simulink model "GFo_29bus"  (R2017b)
settings: Solver=ode1  StartTime=0.0  StopTime=4.5  FixedStep=Time_Step  RelTol=1e-3  EnableMultiTasking=on
PreLoadFcn:
  | Init_29bus;
InitFcn:
  | Init_29bus;
undefined symbols (not defined in the file): D1, D11, Delta, Time_Step, VSC01_Delta_P_Time_Step, VSC01_Delta_P_Value
libraries: powerlib x168, sps_avr x6, GFo_Lib x1
(part 2 of 5)

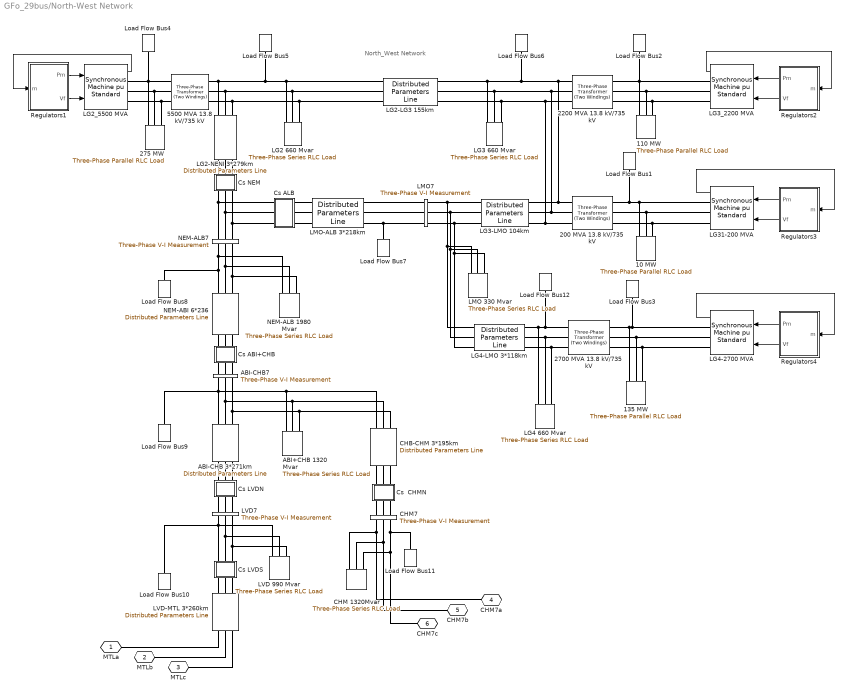
== system GFo_29bus/North-West Network ==
  note: North_West Network
  10 MW : powerlib/Elements/Three-Phase Parallel RLC Load  LConnTagsString=A|B|C  Configuration=Y (grounded)  NominalVoltage=(13800)*1  Vabc=[1e3 1e3 1e3]  Vabcp=[1e3 1e3 1e3]  NominalFrequency=60  UnbalancedPower=off  ActivePower=10000000  InductivePower=0  CapacitivePower=0  Pabc=[10e3 9e3 11e3]  QLabc=[100 90 110]  QCabc=[100 90 110]  Pabcp=[10e3 9e3 11e3]  QLabcp=[100 90 110]  QCabcp=[100 90 110]  Measurements=None  LoadType=constant PQ
  110 MW : powerlib/Elements/Three-Phase Parallel RLC Load  LConnTagsString=A|B|C  Configuration=Y (grounded)  NominalVoltage=(13800)*1  Vabc=[1e3 1e3 1e3]  Vabcp=[1e3 1e3 1e3]  NominalFrequency=60  UnbalancedPower=off  ActivePower=110000000  InductivePower=0  CapacitivePower=0  Pabc=[10e3 9e3 11e3]  QLabc=[100 90 110]  QCabc=[100 90 110]  Pabcp=[10e3 9e3 11e3]  QLabcp=[100 90 110]  QCabcp=[100 90 110]  Measurements=None  LoadType=constant PQ
  135 MW : powerlib/Elements/Three-Phase Parallel RLC Load  LConnTagsString=A|B|C  Configuration=Y (grounded)  NominalVoltage=(13800)*1  Vabc=[1e3 1e3 1e3]  Vabcp=[1e3 1e3 1e3]  NominalFrequency=60  UnbalancedPower=off  ActivePower=135000000  InductivePower=0  CapacitivePower=0  Pabc=[10e3 9e3 11e3]  QLabc=[100 90 110]  QCabc=[100 90 110]  Pabcp=[10e3 9e3 11e3]  QLabcp=[100 90 110]  QCabcp=[100 90 110]  Measurements=None  LoadType=constant PQ
  200 MVA 13.8 kV/735 kV : powerlib/Elements/Three-Phase Transformer (Two Windings)  Winding1Connection=Delta (D1)  Winding2Connection=Yg  CoreType=Three single-phase transformers  SetSaturation=off  Hysteresis=off  DataFile='basic_model'  SetInitialFlux=off  Measurements=None  UNITS=pu  NominalPower=[ 200e6 60 ]  Winding1="[ 13.8e3 0.002  0.0]"  Winding2=[ 735e3 0.002 0.12]  Rm=500  Lm=500  L0=0.5  Saturation="[ 0,0  ;  0.005,1.2  ;  1.0,1.4 ]"  InitialFluxes=[ 0.8 , -0.8 , 0.7 ]  MoreParameters=off  BreakLoop=off  DataType=off  TransfoNumber=0
  2200 MVA 13.8 kV/735 kV : powerlib/Elements/Three-Phase Transformer (Two Windings)  Winding1Connection=Delta (D1)  Winding2Connection=Yg  CoreType=Three single-phase transformers  SetSaturation=off  Hysteresis=off  DataFile='basic_model'  SetInitialFlux=off  Measurements=None  UNITS=pu  NominalPower=[ 2200e6 60 ]  Winding1="[ 13.8e3 0.002  0.0]"  Winding2=[ 735e3 0.002 0.12]  Rm=500  Lm=500  L0=0.5  Saturation="[ 0,0  ;  0.005,1.2  ;  1.0,1.4 ]"  InitialFluxes=[ 0.8 , -0.8 , 0.7 ]  MoreParameters=off  BreakLoop=off  DataType=off  TransfoNumber=0
  2700 MVA 13.8 kV/735 kV : powerlib/Elements/Three-Phase Transformer (Two Windings)  Winding1Connection=Delta (D1)  Winding2Connection=Yg  CoreType=Three single-phase transformers  SetSaturation=off  Hysteresis=off  DataFile='basic_model'  SetInitialFlux=off  Measurements=None  UNITS=pu  NominalPower=[ 2700e6 60 ]  Winding1="[ 13.8e3 0.002  0.0]"  Winding2=[ 735e3 0.002 0.12]  Rm=500  Lm=500  L0=0.5  Saturation="[ 0,0  ;  0.005,1.2  ;  1.0,1.4 ]"  InitialFluxes=[ 0.8 , -0.8 , 0.7 ]  MoreParameters=off  BreakLoop=off  DataType=off  TransfoNumber=0
  275 MW : powerlib/Elements/Three-Phase Parallel RLC Load  LConnTagsString=A|B|C  Configuration=Y (grounded)  NominalVoltage=(13800)*1  Vabc=[1e3 1e3 1e3]  Vabcp=[1e3 1e3 1e3]  NominalFrequency=60  UnbalancedPower=off  ActivePower=275000000  InductivePower=0  CapacitivePower=0  Pabc=[10e3 9e3 11e3]  QLabc=[100 90 110]  QCabc=[100 90 110]  Pabcp=[10e3 9e3 11e3]  QLabcp=[100 90 110]  QCabcp=[100 90 110]  Measurements=None  LoadType=constant PQ
  5500 MVA 13.8 kV/735 kV : powerlib/Elements/Three-Phase Transformer (Two Windings)  Winding1Connection=Delta (D1)  Winding2Connection=Yg  CoreType=Three single-phase transformers  SetSaturation=off  Hysteresis=off  DataFile='basic_model'  SetInitialFlux=off  Measurements=None  UNITS=pu  NominalPower=[ 5500e6 60 ]  Winding1="[ 13.8e3 0.002  0.0]"  Winding2=[ 735e3 0.002 0.12]  Rm=500  Lm=500  L0=0.5  Saturation="[ 0,0  ;  0.005,1.2  ;  1.0,1.4 ]"  InitialFluxes=[ 0.8 , -0.8 , 0.7 ]  MoreParameters=off  BreakLoop=off  DataType=off  TransfoNumber=0
  ABI+CHB 1320 Mvar : powerlib/Elements/Three-Phase Series RLC Load  LConnTagsString=A|B|C  Configuration=Y (grounded)  NominalVoltage=735e3  Vabc=[1e3 1e3 1e3]  Vabcp=[1e3 1e3 1e3]  NominalFrequency=60  UnbalancedPower=off  ActivePower=4400000  InductivePower=1320e6  CapacitivePower=0  Pabc=[10e3 9e3 11e3]  QLabc=[100 90 110]  QCabc=[100 90 110]  Pabcp=[10e3 9e3 11e3]  QLabcp=[100 90 110]  QCabcp=[100 90 110]  Measurements=None  LoadType=constant Z
  ABI-CHB 3*271km : powerlib/Elements/Distributed Parameters Line  Phases=3  Frequency=60  Resistance="[0.01273  0.3864]/3"  Inductance="[0.9337e-3  4.1264e-3]/3"  Capacitance=[12.74e-9 7.751e-9]*3  Length=271  x1=[-0.00156 -3.8452560916682e-08 0 0;-0.00152 -3.64189744128759e-08 0 0;-0.00148 -3.43771065483522e-08 0 0;-0.00144 -3.2327421626255e-08 0 0;-0.0014 -3.02703857272598e-08 0 0;-0.00136 -2.82064666035909e-08 0 0;-0.00132 -2.61361335726585e-08 0 0;-0.00128 -2.40598574103402e-08 0 0;-0.00124 -2.19781102439301e-08 0 0;-0.0012 -1.98913654447816e-08 0 0;-0.00116 -1.78000975206669e-08 0 0;-0.00112 -1.57047820078775e-08 0 0;-0.00108 -1.36058953630917e-08 0 0;-0.00104 -1.15039148550326e-08 0 0;-0.001 -9.39931845594105e-09 0 0;-0.00096 -7.29258473288888e-09 123121.325667195 -796454.043668796;-0.00092 -5.18419273895701e-09 135117.082377557 -794506.987955466;-0.00088 -3.07462190430287e-09 147082.114628586 -792379.268204613;-0.00084 -9.6435192714211e-10 159013.701675131 -790071.368241357;-0.0008 1.14613733533067e-09 170909.130377191 -787583.812862248;-0.00076 3.25636597605726e-09 182765.69581686 -784917.167715928;-0.00072 5.3658541472426e-09 194580.701913405 -782072.039174507;-0.00068 7.47412216946802e-09 206351.462036328 -779049.07419568;-0.00064 9.58069064076618e-09 218075.299616282 -775848.960175613;-0.0006 1.1685080545633e-08 229749.548753705 -772472.424792639;-0.00056 1.37868133639516e-08 241371.554825018 -768920.235841786;-0.00052 1.58854111798036e-08 252938.675086262 -765193.201060188;-0.00048 1.79803967901433e-08 264448.279274042 -761292.167943414;-0.00044 2.00712938133092e-08 275897.750203621 -757218.023552754;-0.0004 2.21576267973495e-08 287284.484364043 -752971.694313508;-0.00036 2.42389213281353e-08 298605.892510158 -748554.145804326;-0.00032 2.63147041372386e-08 309859.400251383 -743966.382537645;-0.00028 2.83845032095495e-08 321042.448637104 -739209.447731267;-0.00024 3.0447847890608e-08 332152.494738558 -734284.423071146;-0.0002 3.25042689936273e-08 343187.012227069 -729192.428465418;-0.00016 3.45532989061823e-08 354143.491948518 -723934.621789744;-0.00012 3.6594471696541e-08 365019.442493902 -718512.198624022;-8e-05 3.86273232196132e-08 375812.390765856 -712926.391980518;-4e-05 4.0651391222493e-08 386519.882541018 -707178.472023493]  x2=[-0.00156 -7.69394572937684e-08 0 0;-0.00152 -7.25740724890193e-08 0 0;-0.00148 -6.81921849660384e-08 0 0;-0.00144 -6.37947911282605e-08 0 0;-0.0014 -5.93828909051229e-08 0 0;-0.00136 -5.49574875246898e-08 0 0;-0.00132 -5.05195872855267e-08 0 0;-0.00128 -4.60701993278772e-08 0 0;-0.00124 -4.16103354041931e-08 0 0;-0.0012 -3.71410096490703e-08 0 0;-0.00116 -3.26632383486437e-08 0 0;-0.00112 -2.81780397094924e-08 0 0;-0.00108 -2.36864336271083e-08 0 0;-0.00104 -1.91894414539804e-08 0 0;-0.001 -1.46880857673486e-08 0 0;-0.00096 -1.0183390136678e-08 -123389.155033361 -813372.162639077;-0.00092 -5.67637889090808e-09 -111110.252745338 -815140.324111655;-0.00088 -1.16807688552937e-09 -98806.084944014 -816723.129704001;-0.00084 3.34049073046001e-09 -86479.4494910415 -818120.219499772;-0.0008 7.84829874766446e-09 -74133.1493570218 -819331.275812798;-0.00076 1.23543221294145e-08 -61769.9919841353 -820356.023259316;-0.00072 1.68575362448515e-08 -49392.7886477534 -821194.228820593;-0.00068 2.13569171019196e-08 -37004.3538171782 -821845.701895914;-0.00064 2.5851441580213e-08 -24607.504515657 -822310.29434592;-0.0006 3.03400876636243e-08 -12205.059679815 -822587.900526293;-0.00056 3.48218346727427e-08 200.160481346233 -822678.457311783;-0.00052 3.92956634969472e-08 12605.3351277401 -822581.944110556;-0.00048 4.37605568261439e-08 25007.6434296298 -822298.382868884;-0.00044 4.82154993820933e-08 37404.2652090602 -821827.838066146;-0.0004 5.2659478149276e-08 49792.3815811428 -821170.416700174;-0.00036 5.70914826052435e-08 62169.175595045 -820326.268262915;-0.00032 6.15105049504026e-08 74531.8328745411 -819295.584706447;-0.00028 6.59155403371799e-08 86877.5422579766 -818078.60039932;-0.00024 7.0305587098516e-08 99203.4964375027 -816675.592073272;-0.0002 7.46796469756355e-08 111506.892597433 -815086.878760297;-0.00016 7.90367253450425e-08 123784.933051582 -813312.821720102;-0.00012 8.33758314446898e-08 136034.82587943 -811353.824357958;-8e-05 8.7695978599269e-08 148253.785560988 -809210.332132973;-4e-05 9.19961844445728e-08 160439.033610196 -806882.832456794]  x3=[-0.00156 -1.37891885995195e-09 0 0;-0.00152 -1.3722422723815e-09 0 0;-0.00148 -1.36525364875204e-09 0 0;-0.00144 -1.35795457821629e-09 0 0;-0.0014 -1.35034672051995e-09 0 0;-0.00136 -1.34243180562426e-09 0 0;-0.00132 -1.33421163331262e-09 0 0;-0.00128 -1.32568807278131e-09 0 0;-0.00124 -1.31686306221449e-09 0 0;-0.0012 -1.30773860834347e-09 0 0;-0.00116 -1.29831678599038e-09 0 0;-0.00112 -1.28859973759635e-09 0 0;-0.00108 -1.27858967273441e-09 0 0;-0.00104 -1.26828886760697e-09 0 0;-0.001 -1.2576996645283e-09 0 0;-0.00096 -1.24682447139185e-09 -1025.79722603647 -1146.3924319426;-0.00092 -1.23566576112277e-09 -1008.39460171361 -1161.73052146923;-0.00088 -1.22422607111553e-09 -990.762677154345 -1176.80444349362;-0.00084 -1.212508002657e-09 -972.90546170627 -1191.61077033589;-0.0008 -1.20051422033489e-09 -954.827015946182 -1206.146135165;-0.00076 -1.18824745143186e-09 -936.531450756745 -1220.40723276433;-0.00072 -1.17571048530539e-09 -918.02292639171 -1234.39082028327;-0.00068 -1.16290617275346e-09 -899.305651529905 -1248.09371797462;-0.00064 -1.14983742536632e-09 -880.383882318225 -1261.5128099176;-0.0006 -1.13650721486443e-09 -861.261921403812 -1274.64504472642;-0.00056 -1.1229185724227e-09 -841.944116955679 -1287.48743624415;-0.00052 -1.10907458798123e-09 -822.434861675967 -1300.03706422169;-0.00048 -1.09497840954271e-09 -802.738591801085 -1312.29107498188;-0.00044 -1.08063324245656e-09 -782.859786092952 -1324.24668206832;-0.0004 -1.06604234869005e-09 -762.802964820555 -1335.90116687908;-0.00036 -1.05120904608661e-09 -742.572688732092 -1347.25187928482;-0.00032 -1.03613670761132e-09 -722.173558017884 -1358.29623823141;-0.00028 -1.02082876058399e-09 -701.610211264343 -1369.03173232688;-0.00024 -1.00528868589976e-09 -680.88732439919 -1379.45592041244;-0.0002 -9.89520017237592e-10 -660.00960962819 -1389.56643211762;-0.00016 -9.73526340256762e-10 -638.981814363641 -1399.36096839924;-0.00012 -9.57311291781491e-10 -617.80872014485 -1408.83730206423;-8e-05 -9.40878558973969e-10 -596.495141550854 -1417.99327827602;-4e-05 -9.24231878495929e-10 -575.045925105624 -1426.82681504459]  x4=[-0.00156 4.69352936032902e-10 0 0;-0.00152 4.84294936998338e-10 0 0;-0.00148 4.99126813471482e-10 0 0;-0.00144 5.13845192811529e-10 0 0;-0.0014 5.28446728185943e-10 0 0;-0.00136 5.42928099331498e-10 0 0;-0.00132 5.57286013309277e-10 0 0;-0.00128 5.7151720525346e-10 0 0;-0.00124 5.85618439113723e-10 0 0;-0.0012 5.99586508391089e-10 0 0;-0.00116 6.13418236867062e-10 0 0;-0.00112 6.27110479325864e-10 0 0;-0.00108 6.40660122269638e-10 0 0;-0.00104 6.54064084626425e-10 0 0;-0.001 6.67319318450777e-10 0 0;-0.00096 6.8042280961683e-10 -2132.85907292929 -16521.1252471031;-0.00092 6.93371578503692e-10 -1883.49323206401 -16551.4092311591;-0.00088 7.06162680672985e-10 -1633.69910108033 -16577.9295674892;-0.00084 7.1879320753838e-10 -1383.53348100947 -16600.6802255976;-0.0008 7.31260287026989e-10 -1133.05325735612 -16619.6560321809;-0.00076 7.43561084232449e-10 -882.315387163084 -16634.8526723043;-0.00072 7.55692802059552e-10 -631.376886059769 -16646.2666903828;-0.00068 7.67652681860283e-10 -380.294815297326 -16653.8954909673;-0.00064 7.79438004061115e-10 -129.126268773408 -16657.7373393341;-0.0006 7.9104608878141e-10 122.071639950492 -16657.7913618803;-0.00056 8.02474296442807e-10 373.241790636168 -16654.0575463214;-0.00052 8.13720028369436e-10 624.327069357354 -16646.5367416949;-0.00048 8.24780727378837e-10 875.270381486935 -16635.230658167;-0.00044 8.35653878363439e-10 1126.01466467978 -16620.1418666436;-0.0004 8.46337008862472e-10 1376.50290184821 -16601.2737981857;-0.00036 8.5682768962419e-10 1626.67813412721 -16578.6307432293;-0.00032 8.67123535158254e-10 1876.48347382639 -16552.21785061;-0.00028 8.77222204278178e-10 2125.86211736573 -16522.0411263917;-0.00024 8.87121400633692e-10 2374.75735819223 -16488.1074325012;-0.0002 8.9681887323291e-10 2623.11259967451 -16450.424485168;-0.00016 9.06312416954192e-10 2870.87136797239 -16409.0008531693;-0.00012 9.15599873047564e-10 3117.97732487853 -16363.8459558818;-8e-05 9.24679129625602e-10 3364.37428062928 -16314.9700611397;-4e-05 9.33548122143656e-10 3610.00620668175 -16262.3842829]  x5=0.00153261764655846  V1=ones(3,3)  V2=ones(3,3)  I1=ones(3,3)  I2=ones(3,3)  nHarmo=1  Measurements=None
      settings: AttributesFormatString=\n  SourceProductName=Simscape Power Systems
  ABI-CHB7 : powerlib/Measurements/Three-Phase V-I Measurement  VoltageMeasurement=no  SetLabelV=on  LabelV=Vabc_ABI7  Vpu=on  VpuLL=off  CurrentMeasurement=no  SetLabelI=off  LabelI=A1  Ipu=off  Pbase=100e6  Vbase=500e3  OutputType=Magnitude  PhasorSimulation=off  PSBequivalent=0
  CHB-CHM 3*195km : powerlib/Elements/Distributed Parameters Line  Phases=3  Frequency=60  Resistance="[0.01273  0.3864]/3"  Inductance="[0.9337e-3  4.1264e-3]/3"  Capacitance=[12.74e-9 7.751e-9]*3  Length=195  x1=[-0.00112 -1.57340244697438e-08 0 0;-0.00108 -1.36362948191761e-08 0 0;-0.00104 -1.15354643927609e-08 0 0;-0.001 -9.43201090122036e-09 0 0;-0.00096 -7.32641265173913e-09 0 0;-0.00092 -5.21914843920118e-09 0 0;-0.00088 -3.11069743731617e-09 0 0;-0.00084 -1.00153908965942e-09 0 0;-0.0008 1.1078469993494e-09 0 0;-0.00076 3.21698117350424e-09 0 0;-0.00072 5.32538383388229e-09 0 0;-0.00068 7.43257554790067e-09 206351.462036328 -779049.07419568;-0.00064 9.53807715833526e-09 218075.299616282 -775848.960175613;-0.0006 1.16414098922769e-08 229749.548753705 -772472.424792639;-0.00056 1.37420954700003e-08 241371.554825018 -768920.235841786;-0.00052 1.58396562137206e-08 252938.675086262 -765193.201060188;-0.00048 1.79336151562133e-08 264448.279274042 -761292.167943414;-0.00044 2.00234961492724e-08 275897.750203621 -757218.023552754;-0.0004 2.21088239719824e-08 287284.484364043 -752971.694313508;-0.00036 2.41891244387795e-08 298605.892510158 -748554.145804326;-0.00032 2.62639245072774e-08 309859.400251383 -743966.382537645;-0.00028 2.83327523858328e-08 321042.448637104 -739209.447731267;-0.00024 3.03951376408269e-08 332152.494738558 -734284.423071146;-0.0002 3.24506113036379e-08 343187.012227069 -729192.428465418;-0.00016 3.44987059772807e-08 354143.491948518 -723934.621789744;-0.00012 3.65389559426884e-08 365019.442493902 -718512.198624022;-8e-05 3.85708972646133e-08 375812.390765856 -712926.391980518;-4e-05 4.05940678971215e-08 386519.882541018 -707178.472023493]  x2=[-0.00112 -6.77914093750269e-09 0 0;-0.00108 -5.32034013604767e-09 0 0;-0.00104 -3.86032953512641e-09 0 0;-0.001 -2.3994411285589e-09 0 0;-0.00096 -9.38007109770666e-10 0 0;-0.00092 5.23640203745304e-10 0 0;-0.00088 1.98516844599463e-09 0 0;-0.00084 3.4462452780587e-09 0 0;-0.0008 4.90653846366568e-09 0 0;-0.00076 6.36571594473822e-09 0 0;-0.00072 7.82344591690052e-09 0 0;-0.00068 9.27939690492784e-09 118695.788002337 -793597.57910968;-0.00064 1.07332378381211e-08 130648.969041902 -791717.567766348;-0.0006 1.21846381255895e-08 142572.441632576 -789657.526675586;-0.00056 1.36332677314239e-08 154463.494479515 -787417.924272976;-0.00052 1.50787972497445e-08 166319.423659846 -784999.269824789;-0.00048 1.65208979796045e-08 178137.533237514 -782402.113312189;-0.00044 1.79592419997342e-08 189915.135876316 -779627.04530617;-0.0004 1.9393502243107e-08 201649.553450979 -776674.696833266;-0.00036 2.08233525713121e-08 213338.117656138 -773545.739232059;-0.00032 2.22484678487155e-08 224978.170613092 -770240.884000526;-0.00028 2.36685240163927e-08 236567.065474178 -766760.882634245;-0.00024 2.50831981658172e-08 248102.167024643 -763106.526455517;-0.0002 2.64921686122871e-08 259580.852281868 -759278.646433424;-0.00016 2.78951149680733e-08 271000.511091814 -755278.112994872;-0.00012 2.9291718215273e-08 282358.546722546 -751105.835826666;-8e-05 3.06816607783516e-08 293652.376454711 -746762.763668654;-4e-05 3.20646265963565e-08 304879.432168819 -742249.884097991]  x3=[-0.00112 2.33399313420562e-10 0 0;-0.00108 2.41014554085093e-10 0 0;-0.00104 2.48574990118446e-10 0 0;-0.001 2.56078902342666e-10 0 0;-0.00096 2.63524584432823e-10 0 0;-0.00092 2.7091034330502e-10 0 0;-0.00088 2.7823449950138e-10 0 0;-0.00084 2.85495387571946e-10 0 0;-0.0008 2.92691356453385e-10 0 0;-0.00076 2.9982076984443e-10 0 0;-0.00072 3.06882006577956e-10 0 0;-0.00068 3.13873460989624e-10 399.328451062111 -5036.75917956306;-0.00064 3.20793543282992e-10 475.231927360191 -5030.16562723451;-0.0006 3.27640679891024e-10 551.027340016215 -5022.42825862063;-0.00056 3.34413313833901e-10 626.697453806977 -5013.54883313232;-0.00052 3.4110990507307e-10 702.225062001152 -5003.52936987436;-0.00048 3.47728930861432e-10 777.592990271958 -4992.37214718629;-0.00044 3.54268886089603e-10 852.784100602454 -4980.07970212433;-0.0004 3.60728283628161e-10 927.781295182568 -4966.65482988449;-0.00036 3.67105654665811e-10 1002.567520297 -4952.10058316694;-0.00032 3.73399549043374e-10 1077.1257702031 -4936.42027148187;-0.00028 3.79608535583546e-10 1151.43909099779 -4919.61746039695;-0.00024 3.8573120241633e-10 1225.49058447277 -4901.6959707265;-0.0002 3.91766157300088e-10 1299.26341195702 -4882.65987766274;-0.00016 3.97712027938125e-10 1372.74079814577 -4862.51350984906;-0.00012 4.0356746229073e-10 1445.90603491502 -4841.26144839577;-8e-05 4.09331128882629e-10 1518.74248512091 -4818.90852583838;-4e-05 4.1500171710574e-10 1591.23358638275 -4795.45982503871]  x4=[-0.00112 -5.12172901448853e-10 0 0;-0.00108 -5.06547662638855e-10 0 0;-0.00104 -5.00807239258654e-10 0 0;-0.001 -4.94952936631024e-10 0 0;-0.00096 -4.88986085973895e-10 0 0;-0.00092 -4.82908044097653e-10 0 0;-0.00088 -4.76720193096604e-10 0 0;-0.00084 -4.70423940034705e-10 0 0;-0.0008 -4.64020716625606e-10 0 0;-0.00076 -4.57511978907089e-10 0 0;-0.00072 -4.50899206909985e-10 0 0;-0.00068 -4.44183904321619e-10 966.84418643773 -12727.6275437189;-0.00064 -4.37367598143889e-10 1158.65512674327 -12711.6018358708;-0.0006 -4.30451838346038e-10 1350.2025988648 -12692.6856193854;-0.00056 -4.23438197512206e-10 1541.443046559 -12670.8831956472;-0.00052 -4.16328270483835e-10 1732.33298339725 -12646.1995223393;-0.00048 -4.09123673997018e-10 1922.82900265409 -12618.6402123163;-0.00044 -4.01826046314867e-10 2112.88778717749 -12588.2115323274;-0.0004 -3.94437046854984e-10 2302.46611923885 -12554.9204015923;-0.00036 -3.86958355812126e-10 2491.52089036032 -12518.7743902268;-0.00032 -3.79391673776144e-10 2680.00911111728 -12479.7817175223;-0.00028 -3.71738721345279e-10 2867.88792091379 -12437.9512500763;-0.00024 -3.64001238734918e-10 3055.1145977287 -12393.2924997764;-0.0002 -3.56180985381882e-10 3241.64656783027 -12345.8156216372;-0.00016 -3.48279739544345e-10 3427.44141545708 -12295.5314114914;-0.00012 -3.40299297897471e-10 3612.45689246302 -12242.4513035349;-8e-05 -3.32241475124872e-10 3796.65092792411 -12186.5873677262;-4e-05 -3.24108103505957e-10 3979.98163770511 -12127.9523070429]  x5=0.0011028060556417  V1=ones(3,3)  V2=ones(3,3)  I1=ones(3,3)  I2=ones(3,3)  nHarmo=1  Measurements=None
      settings: AttributesFormatString=\n  SourceProductName=Simscape Power Systems
  CHM 1320Mvar : powerlib/Elements/Three-Phase Series RLC Load  LConnTagsString=A|B|C  Configuration=Y (grounded)  NominalVoltage=735e3  Vabc=[1e3 1e3 1e3]  Vabcp=[1e3 1e3 1e3]  NominalFrequency=60  UnbalancedPower=off  ActivePower=4400000  InductivePower=1320e6  CapacitivePower=0  Pabc=[10e3 9e3 11e3]  QLabc=[100 90 110]  QCabc=[100 90 110]  Pabcp=[10e3 9e3 11e3]  QLabcp=[100 90 110]  QCabcp=[100 90 110]  Measurements=None  LoadType=constant Z
  CHM7 : powerlib/Measurements/Three-Phase V-I Measurement  VoltageMeasurement=no  SetLabelV=on  LabelV=Vabc_CHM7  Vpu=on  VpuLL=off  CurrentMeasurement=no  SetLabelI=off  LabelI=A1  Ipu=off  Pbase=100e6  Vbase=735e3  OutputType=Magnitude  PhasorSimulation=off  PSBequivalent=0
  "Cs  CHMN " : Subsystem  mask{Xc=25/3}
      mask prompts: Xc "Condensator Reactance at  60Hz  (ohm):"
      mask help: Series Compensation
      mask init:
      | Cs=1/Xc/(2*pi*60);
      mask Display: disp('Cs')
  "Cs ABI+CHB " : Subsystem  mask{Xc=25/6}
      mask prompts: Xc "Condensator Reactance at  60Hz  (ohm):"
      mask help: Series Compensation
      mask init:
      | Cs=1/Xc/(2*pi*60);
      mask Display: disp('Cs')
  Cs ALB : Subsystem  mask{Xc=16/3}
      mask prompts: Xc "Reactance @ 60Hz du condensateur (ohm):"
      mask init:
      | Cs=1/Xc/(2*pi*60);
      mask Display: disp('Cs')
  "Cs LVDN " : Subsystem  mask{Xc=34/3}
      mask prompts: Xc "Condensator Reactance at  60Hz  (ohm):"
      mask help: Series Compensation
      mask init:
      | Cs=1/Xc/(2*pi*60);
      mask Display: disp('Cs')
  "Cs LVDS " : Subsystem  mask{Xc=34/3}
      mask prompts: Xc "Condensator Reactance at  60Hz  (ohm):"
      mask help: Series Compensation
      mask init:
      | Cs=1/Xc/(2*pi*60);
      mask Display: disp('Cs')
  "Cs NEM " : Subsystem  mask{Xc=16/3}
      mask prompts: Xc "Condensator Reactance at  60Hz  (ohm):"
      mask help: Series Compensation
      mask init:
      | Cs=1/Xc/(2*pi*60);
      mask Display: disp('Cs')
  LG2 660 Mvar : powerlib/Elements/Three-Phase Series RLC Load  LConnTagsString=A|B|C  Configuration=Y (grounded)  NominalVoltage=735e3  Vabc=[1e3 1e3 1e3]  Vabcp=[1e3 1e3 1e3]  NominalFrequency=60  UnbalancedPower=off  ActivePower=2200000  InductivePower=660e6  CapacitivePower=0  Pabc=[10e3 9e3 11e3]  QLabc=[100 90 110]  QCabc=[100 90 110]  Pabcp=[10e3 9e3 11e3]  QLabcp=[100 90 110]  QCabcp=[100 90 110]  Measurements=None  LoadType=constant Z
  LG2-LG3 155km : powerlib/Elements/Distributed Parameters Line  Phases=3  Frequency=60  Resistance="[0.01273  0.3864]"  Inductance="[0.9337e-3  4.1264e-3]"  Capacitance=[12.74e-9 7.751e-9]  Length=155  x1=[-0.00088 -1.9399100123935e-09 415587.672863184 -614459.217668148;-0.00084 -1.83186752142981e-09 424805.862965605 -608122.737717224;-0.0008 -1.72340847958909e-09 433927.455878156 -601647.975899972;-0.00076 -1.61455754952216e-09 442950.377429272 -595036.40452139;-0.00072 -1.50533948299182e-09 451872.575884402 -588289.526995796;-0.00068 -1.39577911524454e-09 460692.022412559 -581408.877504956;-0.00064 -1.28590135936314e-09 469406.711547658 -574396.020649228;-0.0006 -1.17573120060176e-09 478014.661644543 -567252.551091784;-0.00056 -1.06529369070444e-09 486513.915329592 -559980.093196;-0.00052 -9.54613942208553e-10 494902.539945812 -552580.300656086;-0.00048 -8.43717122734449e-10 503178.627992307 -545054.856121052;-0.00044 -7.32628449262542e-10 511340.297558024 -537405.470812089;-0.0004 -6.21373182399191e-10 519385.692749687 -529633.884133451;-0.00036 -5.09976620632657e-10 527312.98411381 -521741.863276929;-0.00032 -3.98464094580442e-10 535120.369052699 -513731.202820008;-0.00028 -2.86860961229327e-10 542806.072234347 -505603.724317795;-0.00024 -1.75192598169412e-10 550368.34599613 -497361.275888813;-0.0002 -6.34843978234705e-11 557805.470742207 -489005.731794755;-0.00016 4.82382383270702e-11 565115.755334547 -480538.992014292;-0.00012 1.59949905518204e-10 572297.537477475 -471962.981811038;-8e-05 2.71625201480173e-10 579349.184095664 -463279.651295754;-4e-05 3.8323873221372e-10 586269.091705484 -454490.97498292]  x2=[-0.00088 -2.93952786722991e-09 413310.722035332 -609787.007539505;-0.00084 -2.90618950351965e-09 422458.718213806 -603485.390922945;-0.0008 -2.87219029737821e-09 431510.650922886 -597046.546932726;-0.00076 -2.83753797993185e-09 440464.461831136 -590471.939706444;-0.00072 -2.80224043081874e-09 449318.114919169 -583763.064253086;-0.00068 -2.76630567639716e-09 458069.596942624 -576921.446113075;-0.00064 -2.72974188792036e-09 466716.917889958 -569948.641011377;-0.0006 -2.69255737967855e-09 475258.111434959 -562846.234503741;-0.00056 -2.65476060710822e-09 483691.235383871 -555615.841616157;-0.00052 -2.61636016486952e-09 492014.372117033 -548259.106477617;-0.00048 -2.57736478489185e-09 500225.629024926 -540777.701946249;-0.00044 -2.53778333438835e-09 508323.138938541 -533173.329228927;-0.0004 -2.49762481383952e-09 516305.060553954 -525447.717494429;-0.00036 -2.45689835494662e-09 524169.578851022 -517602.623480241;-0.00032 -2.4156132185552e-09 531914.905506105 -509639.831093089;-0.00028 -2.37377879254923e-09 539539.279298715 -501561.151003293;-0.00024 -2.33140458971644e-09 547040.966512001 -493368.420233037;-0.0002 -2.28850024558512e-09 554418.261326982 -485063.501738649;-0.00016 -2.24507551623315e-09 561669.486210437 -476648.283986975;-0.00012 -2.20114027606948e-09 568792.992296359 -468124.680525962;-8e-05 -2.15670451558887e-09 575787.159760895 -459494.629549533;-4e-05 -2.11177833910004e-09 582650.398190678 -450760.093456857]  x3=[-0.00088 1.40286124984699e-11 1382.36701026453 -2367.08434783059;-0.00084 1.40500137891377e-11 1417.90313254797 -2345.97063689771;-0.0008 1.4068220227832e-11 1453.11683588655 -2324.32347247279;-0.00076 1.40832276745657e-11 1488.00011298779 -2302.14777693433;-0.00072 1.40950327167747e-11 1522.54503169531 -2279.44859284429;-0.00068 1.41036326700944e-11 1556.74373679248 -2256.23108180135;-0.00064 1.41090255789694e-11 1590.5884517887 -2232.50052326732;-0.0006 1.41112102170988e-11 1624.07148068763 -2208.26231336657;-0.00056 1.41101860877147e-11 1657.18520973725 -2183.521963659;-0.00052 1.41059534236954e-11 1689.92210916113 -2158.28509988678;-0.00048 1.4098513187512e-11 1722.27473487065 -2132.55746069511;-0.00044 1.40878670710103e-11 1754.23573015773 -2106.34489632727;-0.0004 1.40740174950251e-11 1785.79782736766 -2079.65336729434;-0.00036 1.40569676088308e-11 1816.95384955171 -2052.48894301987;-0.00032 1.40367212894243e-11 1847.69671209911 -2024.85780045966;-0.00028 1.40132831406442e-11 1878.01942434804 -1996.76622269725;-0.00024 1.39866584921233e-11 1907.91509117522 -1968.22059751518;-0.0002 1.3956853398077e-11 1937.37691456383 -1939.22741594245;-0.00016 1.39238746359268e-11 1966.39819514929 -1909.79327077852;-0.00012 1.38877297047588e-11 1994.97233374267 -1879.92485509417;-8e-05 1.38484268236187e-11 2023.09283283127 -1849.62896070956;-4e-05 1.38059749296425e-11 2050.75329805609 -1818.91247664979]  x4=[-0.00088 -2.31758602658944e-11 1207.15321374292 -2438.84076514513;-0.00084 -2.30254032880232e-11 1243.79135626553 -2420.36094489669;-0.0008 -2.28697105320071e-11 1280.14667135972 -2401.33075544169;-0.00076 -2.27088174010359e-11 1316.21089214036 -2381.75452408109;-0.00072 -2.25427604808202e-11 1351.97581791464 -2361.63670228109;-0.00068 -2.23715775312717e-11 1387.43331604688 -2340.98186466088;-0.00064 -2.21953074779168e-11 1422.57532380776 -2319.79470795242;-0.0006 -2.20139904030456e-11 1457.39385020777 -2298.08004993242;-0.00056 -2.18276675365974e-11 1491.88097781428 -2275.84282832687;-0.00052 -2.16363812467851e-11 1526.02886455186 -2253.08809968819;-0.00048 -2.14401750304615e-11 1559.82974548556 -2229.82103824544;-0.00044 -2.12390935032282e-11 1593.27593458653 -2206.04693472775;-0.0004 -2.10331823892903e-11 1626.35982647981 -2181.77119516125;-0.00036 -2.08224885110596e-11 1659.07389817367 -2156.99933963976;-0.00032 -2.0607059778507e-11 1691.41071077033 -2131.7370010696;-0.00028 -2.03869451782684e-11 1723.36291115747 -2105.98992388872;-0.00024 -2.01621947625059e-11 1754.92323368026 -2079.76396276043;-0.0002 -1.99328596375257e-11 1786.08450179352 -2053.06508124213;-0.00016 -1.96989919521576e-11 1816.83962969362 -2025.89935042924;-0.00012 -1.94606448858964e-11 1847.18162392967 -1998.27294757467;-8e-05 -1.92178726368097e-11 1877.10358499387 -1970.19215468419;-4e-05 -1.89707304092132e-11 1906.59870889028 -1941.66335708795]  x5=0.000876589428843401  V1=ones(3,3)  V2=ones(3,3)  I1=ones(3,3)  I2=ones(3,3)  nHarmo=1  Measurements=None
      settings: AttributesFormatString=\n  SourceProductName=Simscape Power Systems
  LG2-NENI 3*279km : powerlib/Elements/Distributed Parameters Line  Phases=3  Frequency=60  Resistance="[0.01273  0.3864]/3"  Inductance="[0.9337e-3  4.1264e-3]/3"  Capacitance=[12.74e-9 7.751e-9]*3  Length=279  x1=[-0.0016 -3.78600842431516e-09 0 0;-0.00156 -3.68954651697759e-09 0 0;-0.00152 -3.59224563857934e-09 0 0;-0.00148 -3.4941279145011e-09 0 0;-0.00144 -3.39521565586717e-09 0 0;-0.0014 -3.29553135447219e-09 0 0;-0.00136 -3.19509767766665e-09 0 0;-0.00132 -3.09393746320256e-09 0 0;-0.00128 -2.99207371404032e-09 0 0;-0.00124 -2.88952959311806e-09 0 0;-0.0012 -2.78632841808456e-09 0 0;-0.00116 -2.68249365599705e-09 0 0;-0.00112 -2.57804891798502e-09 0 0;-0.00108 -2.47301795388118e-09 0 0;-0.00104 -2.36742464682103e-09 0 0;-0.001 -2.26129300781199e-09 387374.587748154 -632624.716893096;-0.00096 -2.15464717027354e-09 396869.907125202 -626711.600299158;-0.00092 -2.04751138454945e-09 406274.981707831 -620655.974891844;-0.00088 -1.9399100123935e-09 415587.672863184 -614459.217668148;-0.00084 -1.83186752142981e-09 424805.862965605 -608122.737717224;-0.0008 -1.72340847958909e-09 433927.455878156 -601647.975899972;-0.00076 -1.61455754952216e-09 442950.377429272 -595036.40452139;-0.00072 -1.50533948299182e-09 451872.575884402 -588289.526995796;-0.00068 -1.39577911524454e-09 460692.022412559 -581408.877504956;-0.00064 -1.28590135936314e-09 469406.711547658 -574396.020649228;-0.0006 -1.17573120060176e-09 478014.661644543 -567252.551091784;-0.00056 -1.06529369070444e-09 486513.915329592 -559980.093196;-0.00052 -9.54613942208553e-10 494902.539945812 -552580.300656086;-0.00048 -8.43717122734449e-10 503178.627992307 -545054.856121052;-0.00044 -7.32628449262542e-10 511340.297558024 -537405.470812089;-0.0004 -6.21373182399191e-10 519385.692749687 -529633.884133451;-0.00036 -5.09976620632657e-10 527312.98411381 -521741.863276929;-0.00032 -3.98464094580442e-10 535120.369052699 -513731.202820008;-0.00028 -2.86860961229327e-10 542806.072234347 -505603.724317795;-0.00024 -1.75192598169412e-10 550368.34599613 -497361.275888813;-0.0002 -6.34843978234705e-11 557805.470742207 -489005.731794755;-0.00016 4.82382383270702e-11 565115.755334547 -480538.992014292;-0.00012 1.59949905518204e-10 572297.537477475 -471962.981811038;-8e-05 2.71625201480173e-10 579349.184095664 -463279.651295754;-4e-05 3.8323873221372e-10 586269.091705484 -454490.97498292]  x2=[-0.0016 -2.53773367978642e-08 0 0;-0.00156 -2.41576511298992e-08 0 0;-0.00152 -2.2932472220394e-08 0 0;-0.00148 -2.17020786644671e-08 0 0;-0.00144 -2.04667502430027e-08 0 0;-0.0014 -1.92267678590307e-08 0 0;-0.00136 -1.79824134738522e-08 0 0;-0.00132 -1.67339700429235e-08 0 0;-0.00128 -1.54817214515146e-08 0 0;-0.00124 -1.42259524501563e-08 0 0;-0.0012 -1.29669485898903e-08 0 0;-0.00116 -1.17049961573371e-08 0 0;-0.00112 -1.04403821095973e-08 0 0;-0.00108 -9.17339400899979e-09 0 0;-0.00104 -7.90431995771264e-09 0 0;-0.001 -6.63344853223105e-09 186560.016005174 -764207.038237137;-0.00096 -5.36106871775765e-09 198062.305996751 -761307.055270302;-0.00092 -4.08746984248973e-09 209519.55832796 -758233.957644331;-0.00088 -2.81294151182847e-09 220929.167718426 -754988.444155123;-0.00084 -1.53777354252519e-09 232288.539721364 -751571.252804457;-0.0008 -2.62255896779531e-10 243595.09131354 -747983.160632178;-0.00076 1.01332138369545e-09 254846.251482627 -744224.983539504;-0.00072 2.2886682436263e-09 266039.461811827 -740297.576103495;-0.00068 3.56349468013518e-09 277172.177061637 -736201.831382735;-0.00064 4.83751080868407e-09 288241.865748615 -731938.680714252;-0.0006 6.11042692899197e-09 299246.010721014 -727509.093501745;-0.00056 7.3819535909103e-09 310182.109731162 -722914.076995148;-0.00052 8.65180166024132e-09 321047.676004454 -718154.676061587;-0.00048 9.91968238448476e-09 331840.23880482 -713231.972947792;-0.00044 1.11853074584977e-08 342557.34399655 -708147.087033999;-0.0004 1.24483890900525e-08 353196.554602343 -702901.174579415;-0.00036 1.37086400652786e-08 363755.451357458 -697495.428459293;-0.00032 1.49657738139721e-08 374231.633259827 -691931.077893684;-0.00028 1.62195044747596e-08 384622.71811603 -686209.388167922;-0.00024 1.74695469601007e-08 394926.343082977 -680331.660344907;-0.0002 1.87156170211139e-08 405140.165205208 -674299.230969261;-0.00016 1.99574313122132e-08 415261.86194765 -668113.471763401;-0.00012 2.11947074555377e-08 425289.131723752 -661775.789315628;-8e-05 2.24271641051621e-08 435219.694418837 -655287.624760275;-4e-05 2.36545210110726e-08 445051.291908585 -648650.453450012]  x3=[-0.0016 -5.32321742399182e-10 0 0;-0.00156 -5.32398446695501e-10 0 0;-0.00152 -5.32354088176249e-10 0 0;-0.00148 -5.32188676928172e-10 0 0;-0.00144 -5.31902250564362e-10 0 0;-0.0014 -5.31494874215702e-10 0 0;-0.00136 -5.30966640516063e-10 0 0;-0.00132 -5.30317669581231e-10 0 0;-0.00128 -5.29548108981602e-10 0 0;-0.00124 -5.28658133708619e-10 0 0;-0.0012 -5.27647946134983e-10 0 0;-0.00116 -5.26517775968639e-10 0 0;-0.00112 -5.25267880200536e-10 0 0;-0.00108 -5.23898543046192e-10 0 0;-0.00104 -5.22410075881068e-10 0 0;-0.001 -5.20802817169761e-10 -1322.87812147528 -1644.44662260267;-0.00096 -5.19077132389042e-10 -1297.93133189064 -1664.20816884854;-0.00092 -5.17233413944749e-10 -1272.68940391402 -1683.59128850834;-0.00088 -5.15272081082555e-10 -1247.15807734215 -1702.5915740278;-0.00084 -5.1319357979264e-10 -1221.34315777852 -1721.20470490585;-0.0008 -5.10998382708274e-10 -1195.25051531323 -1739.42644867705;-0.00076 -5.08686988998342e-10 -1168.88608318816 -1757.25266187399;-0.00072 -5.06259924253841e-10 -1142.25585644782 -1774.67929096952;-0.00068 -5.03717740368365e-10 -1115.36589057612 -1791.70237329847;-0.00064 -5.01061015412606e-10 -1088.2223001194 -1808.31803795871;-0.0006 -4.98290353502908e-10 -1060.83125729607 -1824.52250669139;-0.00056 -4.95406384663897e-10 -1033.19899059305 -1840.31209474006;-0.00052 -4.92409764685216e-10 -1005.33178334949 -1855.68321168857;-0.00048 -4.89301174972406e-10 -977.235972328016 -1870.63236227747;-0.00044 -4.86081322391961e-10 -948.917946273757 -1885.15614719883;-0.0004 -4.82750939110591e-10 -920.384144461634 -1899.25126386921;-0.00036 -4.79310782428734e-10 -891.641055232116 -1912.91450718063;-0.00032 -4.75761634608353e-10 -862.695214515823 -1926.1427702294;-0.00028 -4.72104302695056e-10 -833.553204347316 -1938.93304502256;-0.00024 -4.6833961833458e-10 -804.221651368397 -1951.28242316192;-0.0002 -4.64468437583683e-10 -774.707225321269 -1963.18809650541;-0.00016 -4.60491640715485e-10 -745.016637531893 -1974.64735780556;-0.00012 -4.564101320193e-10 -715.156639383892 -1985.65760132518;-8e-05 -4.52224839595006e-10 -685.134020783344 -1996.21632342985;-4e-05 -4.47936715142009e-10 -654.955608614814 -2006.3211231572]  x4=[-0.0016 3.21433967572941e-10 0 0;-0.00156 3.25847986814515e-10 0 0;-0.00152 3.30187911033881e-10 0 0;-0.00148 3.34452753369697e-10 0 0;-0.00144 3.38641544033594e-10 0 0;-0.0014 3.42753330530698e-10 0 0;-0.00136 3.46787177876219e-10 0 0;-0.00132 3.50742168808056e-10 0 0;-0.00128 3.54617403995377e-10 0 0;-0.00124 3.5841200224312e-10 0 0;-0.0012 3.62125100692367e-10 0 0;-0.00116 3.65755855016549e-10 0 0;-0.00112 3.69303439613446e-10 0 0;-0.00108 3.72767047792911e-10 0 0;-0.00104 3.76145891960315e-10 0 0;-0.001 3.7943920379563e-10 4799.79088910052 -14840.2883334513;-0.00096 3.82646234428147e-10 5023.02283562982 -14766.2253269997;-0.00092 3.85766254606756e-10 5245.112590083 -14688.8046082473;-0.00088 3.88798554865773e-10 5466.00965116512 -14608.0437819978;-0.00084 3.9174244568627e-10 5685.66378878942 -14523.9612125666;-0.0008 3.94597257652861e-10 5904.02505549923 -14436.5760196051;-0.00076 3.97362341605923e-10 6121.04379782556 -14345.9080737524;-0.00072 4.00037068789211e-10 6336.6706675779 -14251.9779921176;-0.00068 4.0262083099283e-10 6550.85663306555 -14154.8071335912;-0.00064 4.05113040691534e-10 6763.55299024703 -14054.4175939884;-0.0006 4.07513131178332e-10 6974.71137380492 -13950.832201025;-0.00056 4.09820556693343e-10 7184.28376814376 -13844.0745091259;-0.00052 4.12034792547904e-10 7392.22251830834 -13734.1687940696;-0.00048 4.14155335243876e-10 7598.48034082008 -13621.140047468;-0.00044 4.16181702588137e-10 7803.01033442881 -13505.0139710832;-0.0004 4.18113433802228e-10 8005.7659907778 -13385.8169709838;-0.00036 4.19950089627129e-10 8206.70120497926 -13263.5761515395;-0.00032 4.21691252423144e-10 8405.77028609829 -13138.3193092586;-0.00028 4.23336526264868e-10 8602.92796754254 -13010.0749264668;-0.00024 4.24885537031219e-10 8798.12941735545 -12878.8721648308;-0.0002 4.26337932490506e-10 8991.3302484107 -12744.7408587271;-0.00016 4.27693382380525e-10 9182.48652850539 -12607.7115084582;-0.00012 4.28951578483663e-10 9371.55479034989 -12467.8152733166;-8e-05 4.30112234696974e-10 9558.49204145191 -12325.0839644996;-4e-05 4.31175087097244e-10 9743.25577389262 -12179.5500378761]  x5=0.00157786097191812  V1=ones(3,3)  V2=ones(3,3)  I1=ones(3,3)  I2=ones(3,3)  nHarmo=1  Measurements=None
      settings: AttributesFormatString=\n  SourceProductName=Simscape Power Systems
  LG2_5500 MVA : powerlib/Machines/Synchronous Machine pu Standard  PresetModel=No  MechanicalLoad=Mechanical power Pm  ShowDetailedParameters=on  RotorType=Salient-pole  Units=per unit standard parameters  MeasurementBus=off  NominalParameters="[5500E6  13800   60 ]"  Reactances1=[ 31 32 33 34 35 36 37 ]  Reactances2=[ 1.305, 0.296, 0.252, 0.474, 0.243, 0.18 ]  dAxisTimeConstants=Short-circuit  qAxisTimeConstants=Open-circuit  TimeConstants1=[]  TimeConstants2=[]  TimeConstants3=[]  TimeConstants4=[]  TimeConstants5=[ 1.01, 0.053, 0.1 ]  TimeConstants6=[]  TimeConstants7=[]  TimeConstants8=[]  StatorResistance=2.8544e-3  Mechanical="[ 4.1  0  32]"  PolePairs=32  InitialConditions=[0 -62.7907 1.06459 1.06459 1.06459 2.52703 -117.473 122.527 1.47225]  SetSaturation=off  Saturation=[0.6404,0.7127,0.8441,0.9214,0.9956,1.082,1.19,1.316,1.457;0.7,0.7698,0.8872,0.9466,0.9969,1.046,1.1,1.151,1.201]  LoadFlowParameters=[2 4000000000 0 0 0]  TsPowergui=0  TsBlock=-1  IterativeModel=Trapezoidal non iterative  IterativeDiscreteModel=Trapezoidal non iterative  BusType=swing  Pref=0  Qref=0  Qmin=-Inf  Qmax=Inf  PLF=0  QLF=0
      settings: AttributesFormatString=\n\n  SourceProductName=Simscape Power Systems
  LG3 660 Mvar : powerlib/Elements/Three-Phase Series RLC Load  LConnTagsString=A|B|C  Configuration=Y (grounded)  NominalVoltage=735e3  Vabc=[1e3 1e3 1e3]  Vabcp=[1e3 1e3 1e3]  NominalFrequency=60  UnbalancedPower=off  ActivePower=2200000  InductivePower=660e6  CapacitivePower=0  Pabc=[10e3 9e3 11e3]  QLabc=[100 90 110]  QCabc=[100 90 110]  Pabcp=[10e3 9e3 11e3]  QLabcp=[100 90 110]  QCabcp=[100 90 110]  Measurements=None  LoadType=constant Z
  LG3-LMO 104km : powerlib/Elements/Distributed Parameters Line  Phases=3  Frequency=60  Resistance="[0.01273  0.3864]"  Inductance="[0.9337e-3  4.1264e-3]"  Capacitance=[12.74e-9 7.751e-9]  Length=104  x1=[-0.0006 -2.52238259039188e-09 0 0;-0.00056 -2.48401462679142e-09 0 0;-0.00052 -2.44508181968605e-09 0 0;-0.00048 -2.40559302206038e-09 0 0;-0.00044 -2.36555721332644e-09 0 0;-0.0004 -2.32498349728188e-09 0 0;-0.00036 -2.28388110003985e-09 524169.578851022 -517602.623480241;-0.00032 -2.24225936793102e-09 531914.905506105 -509639.831093089;-0.00028 -2.20012776537834e-09 539539.279298715 -501561.151003293;-0.00024 -2.15749587274492e-09 547040.966512 -493368.420233037;-0.0002 -2.11437338415548e-09 554418.261326982 -485063.501738649;-0.00016 -2.07077010529206e-09 561669.486210437 -476648.283986975;-0.00012 -2.02669595116426e-09 568792.992296359 -468124.680525962;-8e-05 -1.98216094385465e-09 575787.159760895 -459494.629549533;-4e-05 -1.93717521023983e-09 582650.398190678 -450760.093456857]  x2=[-0.0006 2.5677281794813e-09 0 0;-0.00056 3.00776299182222e-09 0 0;-0.00052 3.44711386479664e-09 0 0;-0.00048 3.88568089380485e-09 0 0;-0.00044 4.32336435248649e-09 0 0;-0.0004 4.76006471539748e-09 0 0;-0.00036 5.19568268064125e-09 472944.275465123 -596240.493924388;-0.00032 5.63011919244909e-09 481881.211823625 -589041.193355531;-0.00028 6.06327546370466e-09 490708.572550126 -581707.949898979;-0.00024 6.49505299840723e-09 499424.350378919 -574242.431071057;-0.0002 6.92535361406892e-09 508026.563417289 -566646.334466364;-0.00016 7.35407946404048e-09 516513.255596171 -558921.387371763;-0.00012 7.78113305976079e-09 524882.497114952 -551069.346373608;-8e-05 8.20641729292495e-09 533132.384880283 -543091.996958306;-4e-05 8.62983545756583e-09 541261.04293883 -534991.153106322]  x3=[-0.0006 -1.4780453783326e-10 0 0;-0.00056 -1.46739601869312e-10 0 0;-0.00052 -1.45641298585326e-10 0 0;-0.00048 -1.44509877726e-10 0 0;-0.00044 -1.43345596566678e-10 0 0;-0.0004 -1.42148719854857e-10 0 0;-0.00036 -1.4091951974998e-10 -397.043477365032 -714.736494250849;-0.00032 -1.39658275761549e-10 -386.220858543232 -720.642487277995;-0.00028 -1.38365274685572e-10 -375.310416428827 -726.384612418089;-0.00024 -1.37040810539343e-10 -364.314631962265 -731.961563961394;-0.0002 -1.35685184494587e-10 -353.23600549011 -737.372073757222;-0.00016 -1.34298704808976e-10 -342.077056196484 -742.614911502303;-0.00012 -1.32881686756034e-10 -330.840321530226 -747.688885020547;-8e-05 -1.31434452553447e-10 -319.528356627898 -752.592840534131;-4e-05 -1.29957331289791e-10 -308.143733732767 -757.325662925862]  x4=[-0.0006 1.42426499172884e-10 0 0;-0.00056 1.42017672152751e-10 0 0;-0.00052 1.41576551538678e-10 0 0;-0.00048 1.41103237637689e-10 0 0;-0.00044 1.40597838077285e-10 0 0;-0.0004 1.40060467780965e-10 0 0;-0.00036 1.39491248942102e-10 3788.82122349444 -3633.36443480633;-0.00032 1.38890310996151e-10 3843.17799491343 -3575.81960370957;-0.00028 1.38257790591219e-10 3896.66086079853 -3517.46166207147;-0.00024 1.3759383155699e-10 3949.25765960726 -3458.30387998472;-0.0002 1.36898584872025e-10 4000.95643128115 -3398.35970941881;-0.00016 1.36172208629422e-10 4051.74541996534 -3337.64278116117;-0.00012 1.35414868000876e-10 4101.61307668179 -3276.16690171771;-8e-05 1.34626735199115e-10 4150.54806195541 -3213.94605017326;-4e-05 1.33807989438741e-10 4198.53924839255 -3150.99437501288]  x5=0.000588163229675572  V1=ones(3,3)  V2=ones(3,3)  I1=ones(3,3)  I2=ones(3,3)  nHarmo=1  Measurements=None
      settings: AttributesFormatString=\n  SourceProductName=Simscape Power Systems
  LG31-200 MVA : powerlib/Machines/Synchronous Machine pu Standard  PresetModel=No  MechanicalLoad=Mechanical power Pm  ShowDetailedParameters=on  RotorType=Salient-pole  Units=per unit standard parameters  MeasurementBus=off  NominalParameters="[200E6  13800   60 ]"  Reactances1=[ 31 32 33 34 35 36 37 ]  Reactances2=[ 1.305, 0.296, 0.252, 0.474, 0.243, 0.18 ]  dAxisTimeConstants=Short-circuit  qAxisTimeConstants=Open-circuit  TimeConstants1=[]  TimeConstants2=[]  TimeConstants3=[]  TimeConstants4=[]  TimeConstants5=[ 1.01, 0.053, 0.1 ]  TimeConstants6=[]  TimeConstants7=[]  TimeConstants8=[]  StatorResistance=2.8544e-3  Mechanical="[ 3.2  0  32]"  PolePairs=32  InitialConditions=[0 -67.9718 0.900001 0.900001 0.900001 -0.955416 -120.955 119.045 1.38105]  SetSaturation=off  Saturation=[0.6404,0.7127,0.8441,0.9214,0.9956,1.082,1.19,1.316,1.457;0.7,0.7698,0.8872,0.9466,0.9969,1.046,1.1,1.151,1.201]  LoadFlowParameters=[1 180000000 0 0 0]  TsPowergui=0  TsBlock=-1  IterativeModel=Trapezoidal non iterative  IterativeDiscreteModel=Trapezoidal non iterative  BusType=PV  Pref=180000000  Qref=0  Qmin=-Inf  Qmax=Inf  PLF=0  QLF=0
      settings: AttributesFormatString=\n\n  SourceProductName=Simscape Power Systems
  LG3_2200 MVA : powerlib/Machines/Synchronous Machine pu Standard  PresetModel=No  MechanicalLoad=Mechanical power Pm  ShowDetailedParameters=on  RotorType=Salient-pole  Units=per unit standard parameters  MeasurementBus=off  NominalParameters="[2200E6  13800   60 ]"  Reactances1=[ 31 32 33 34 35 36 37 ]  Reactances2=[ 1.305, 0.296, 0.252, 0.474, 0.243, 0.18 ]  dAxisTimeConstants=Short-circuit  qAxisTimeConstants=Open-circuit  TimeConstants1=[]  TimeConstants2=[]  TimeConstants3=[]  TimeConstants4=[]  TimeConstants5=[ 1.01, 0.053, 0.1 ]  TimeConstants6=[]  TimeConstants7=[]  TimeConstants8=[]  StatorResistance=2.8544e-3  Mechanical="[ 3.2  0  32]"  PolePairs=32  InitialConditions=[0 -70.3849 0.818207 0.818207 0.818207 -1.14608 -121.146 118.854 1.31292]  SetSaturation=off  Saturation=[0.6404,0.7127,0.8441,0.9214,0.9956,1.082,1.19,1.316,1.457;0.7,0.7698,0.8872,0.9466,0.9969,1.046,1.1,1.151,1.201]  LoadFlowParameters=[1 1800000000 0 0 0]  TsPowergui=0  TsBlock=-1  IterativeModel=Trapezoidal non iterative  IterativeDiscreteModel=Trapezoidal non iterative  BusType=PV  Pref=1800000000  Qref=0  Qmin=-Inf  Qmax=Inf  PLF=0  QLF=0
      settings: AttributesFormatString=\n\n  SourceProductName=Simscape Power Systems
  LG4 660 Mvar : powerlib/Elements/Three-Phase Series RLC Load  LConnTagsString=A|B|C  Configuration=Y (grounded)  NominalVoltage=735e3  Vabc=[1e3 1e3 1e3]  Vabcp=[1e3 1e3 1e3]  NominalFrequency=60  UnbalancedPower=off  ActivePower=2200000  InductivePower=660e6  CapacitivePower=0  Pabc=[10e3 9e3 11e3]  QLabc=[100 90 110]  QCabc=[100 90 110]  Pabcp=[10e3 9e3 11e3]  QLabcp=[100 90 110]  QCabcp=[100 90 110]  Measurements=None  LoadType=constant Z
  LG4-2700 MVA : powerlib/Machines/Synchronous Machine pu Standard  PresetModel=No  MechanicalLoad=Mechanical power Pm  ShowDetailedParameters=on  RotorType=Salient-pole  Units=per unit standard parameters  MeasurementBus=off  NominalParameters="[2700E6  13800   60 ]"  Reactances1=[ 31 32 33 34 35 36 37 ]  Reactances2=[ 1.305, 0.296, 0.252, 0.474, 0.243, 0.18 ]  dAxisTimeConstants=Short-circuit  qAxisTimeConstants=Open-circuit  TimeConstants1=[]  TimeConstants2=[]  TimeConstants3=[]  TimeConstants4=[]  TimeConstants5=[ 1.01, 0.053, 0.1 ]  TimeConstants6=[]  TimeConstants7=[]  TimeConstants8=[]  StatorResistance=2.8544e-3  Mechanical="[ 3.7  0  32]"  PolePairs=32  InitialConditions=[0 -69.6741 0.933222 0.933222 0.933222 2.62313 -117.377 122.623 1.28011]  SetSaturation=off  Saturation=[0.6404,0.7127,0.8441,0.9214,0.9956,1.082,1.19,1.316,1.457;0.7,0.7698,0.8872,0.9466,0.9969,1.046,1.1,1.151,1.201]  LoadFlowParameters=[1 2500000000 0 0 0]  TsPowergui=0  TsBlock=-1  IterativeModel=Trapezoidal non iterative  IterativeDiscreteModel=Trapezoidal non iterative  BusType=PV  Pref=2500000000  Qref=0  Qmin=-Inf  Qmax=Inf  PLF=0  QLF=0
      settings: AttributesFormatString=\n\n  SourceProductName=Simscape Power Systems
  LG4-LMO 3*118km : powerlib/Elements/Distributed Parameters Line  Phases=3  Frequency=60  Resistance="[0.01273  0.3864]/3"  Inductance="[0.9337e-3  4.1264e-3]/3"  Capacitance=[12.74e-9 7.751e-9]*3  Length=118  x1=[-0.00068 1.91967558876326e-09 0 0;-0.00064 2.03229981138245e-09 0 0;-0.0006 2.14446190655034e-09 0 0;-0.00056 2.25613636957373e-09 0 0;-0.00052 2.36729780664277e-09 0 0;-0.00048 2.47792094060528e-09 0 0;-0.00044 2.58798061671458e-09 480136.481787822 -572208.501078848;-0.0004 2.69745180834944e-09 488710.222518584 -564903.484105858;-0.00036 2.80630962270491e-09 497172.834759202 -557470.012952103;-0.00032 2.91452930645276e-09 505522.394184633 -549909.777924819;-0.00028 3.02208625137016e-09 513757.002177065 -542224.498156255;-0.00024 3.12895599993535e-09 521874.786257654 -534415.921212755;-0.0002 3.23511425088913e-09 529873.900512304 -526485.822697377;-0.00016 3.34053686476069e-09 537752.526011416 -518436.005846139;-0.00012 3.44519986935677e-09 545508.871223493 -510268.301117973;-8e-05 3.54907946521269e-09 553141.172422522 -501984.5657785;-4e-05 3.65215203100419e-09 560647.694089028 -493586.683477698]  x2=[-0.00068 1.68600710995558e-09 0 0;-0.00064 2.12710948789551e-09 0 0;-0.0006 2.5677281794813e-09 0 0;-0.00056 3.00776299182222e-09 0 0;-0.00052 3.44711386479664e-09 0 0;-0.00048 3.88568089380485e-09 0 0;-0.00044 4.32336435248649e-09 454749.8290356 -610230.74899327;-0.0004 4.76006471539749e-09 463899.795656877 -603304.214546686;-0.00036 5.19568268064125e-09 472944.275465123 -596240.493924388;-0.00032 5.63011919244909e-09 481881.211823625 -589041.193355531;-0.00028 6.06327546370466e-09 490708.572550126 -581707.949898979;-0.00024 6.49505299840723e-09 499424.350378919 -574242.431071057;-0.0002 6.92535361406892e-09 508026.563417289 -566646.334466364;-0.00016 7.35407946404048e-09 516513.255596171 -558921.387371763;-0.00012 7.78113305976079e-09 524882.497114952 -551069.346373608;-8e-05 8.20641729292495e-09 533132.384880283 -543091.996958306;-4e-05 8.62983545756583e-09 541261.04293883 -534991.153106322]  x3=[-0.00068 -3.25084868225663e-10 0 0;-0.00064 -3.23457909689045e-10 0 0;-0.0006 -3.21757399613147e-10 0 0;-0.00056 -3.19983724679293e-10 0 0;-0.00052 -3.1813728820587e-10 0 0;-0.00048 -3.16218510056608e-10 0 0;-0.00044 -3.14227826545111e-10 2000.69388824517 -4987.92594598937;-0.0004 -3.12165690335644e-10 2075.67915698246 -4957.1909097285;-0.00036 -3.10032570340196e-10 2150.19243417934 -4925.32865100374;-0.00032 -3.0782895161186e-10 2224.21677615917 -4892.34641501797;-0.00028 -3.05555335234531e-10 2297.73535042492 -4858.25170164723;-0.00024 -3.03212238208967e-10 2370.73143948682 -4823.0522637353;-0.0002 -3.00800193335225e-10 2443.18844466369 -4786.75610533084;-0.00016 -2.98319749091509e-10 2515.0898898574 -4749.37147986725;-0.00012 -2.9577146950945e-10 2586.41942529937 -4710.90688828598;-8e-05 -2.93155934045848e-10 2657.16083126836 -4671.37107710344;-4e-05 -2.90473737450914e-10 2727.2980217787 -4630.77303642215]  x4=[-0.00068 3.18607960529212e-10 0 0;-0.00064 3.19088195047595e-10 0 0;-0.0006 3.19495871662124e-10 0 0;-0.00056 3.19830897670652e-10 0 0;-0.00052 3.20093196891153e-10 0 0;-0.00048 3.20282709679048e-10 0 0;-0.00044 3.20399392940762e-10 7311.8576763626 -8854.98067266846;-0.0004 3.20443220143528e-10 7444.55093055594 -8743.71842742208;-0.00036 3.20414181321418e-10 7575.55135806674 -8630.46793600792;-0.00032 3.2031228307761e-10 7704.82917052749 -8515.2549506111;-0.00028 3.20137548582886e-10 7832.35497127847 -8398.10566967094;-0.00024 3.19890017570362e-10 7958.09976205234 -8279.04673192367;-0.0002 3.19569746326457e-10 8082.03494956805 -8158.10521034503;-0.00016 3.19176807678089e-10 8204.13235203273 -8035.30860599405;-0.00012 3.18711290976119e-10 8324.36420554998 -7910.68484175962;-8e-05 3.1817330207503e-10 8442.70317043315 -7784.26225601102;-4e-05 3.17562963308859e-10 8559.12233742213 -7656.06959615402]  x5=0.000667339049054976  V1=ones(3,3)  V2=ones(3,3)  I1=ones(3,3)  I2=ones(3,3)  nHarmo=1  Measurements=None
      settings: AttributesFormatString=\n  SourceProductName=Simscape Power Systems
  LMO 330 Mvar : powerlib/Elements/Three-Phase Series RLC Load  LConnTagsString=A|B|C  Configuration=Y (grounded)  NominalVoltage=735e3  Vabc=[1e3 1e3 1e3]  Vabcp=[1e3 1e3 1e3]  NominalFrequency=60  UnbalancedPower=off  ActivePower=1100000  InductivePower=330e6  CapacitivePower=0  Pabc=[10e3 9e3 11e3]  QLabc=[100 90 110]  QCabc=[100 90 110]  Pabcp=[10e3 9e3 11e3]  QLabcp=[100 90 110]  QCabcp=[100 90 110]  Measurements=None  LoadType=constant Z
  LMO-ALB 3*218km : powerlib/Elements/Distributed Parameters Line  Phases=3  Frequency=60  Resistance="[0.01273  0.3864]/3"  Inductance="[0.9337e-3  4.1264e-3]/3"  Capacitance=[12.74e-9 7.751e-9]*3  Length=218  x1=[-0.00124 -4.47086973428242e-09 252961.45706671 -717766.287773167;-0.0012 -4.03392930304985e-09 263755.919912422 -713870.319485688;-0.00116 -3.59607159108089e-09 274490.40693648 -709812.023243713;-0.00112 -3.15739616344331e-09 285162.477209105 -705592.321868811;-0.00108 -2.7180027711464e-09 295769.703993549 -701212.174884685;-0.00104 -2.27799132845838e-09 306309.675297915 -696672.578298986;-0.001 -1.83746189018684e-09 316779.99442362 -691974.564376831;-0.00096 -1.39651462892706e-09 327178.280510387 -687119.20140607;-0.00092 -9.55249812283696e-10 337502.169077631 -682107.593454374;-0.00088 -5.13767780070738e-10 347749.312562122 -676940.880118172;-0.00084 -7.21689214951389e-11 357917.380851799 -671620.23626352;-0.0008 3.69446347670851e-10 368004.061815618 -666146.871758948;-0.00076 8.1097760792335e-10 378007.061829311 -660522.031200344;-0.00072 1.25232445886138e-09 387924.10629694 -654746.993627944;-0.00068 1.69338654201705e-09 397752.940168111 -648823.072235491;-0.00064 2.13406356367621e-09 407491.328450763 -642751.614071624;-0.0006 2.57425531768437e-09 417137.056719381 -636533.99973357;-0.00056 3.01386170823272e-09 426687.931618538 -630171.643053213;-0.00052 3.45278277261906e-09 436141.781361644 -623665.990775594;-0.00048 3.89091870397843e-09 445496.456224796 -617018.522229939;-0.00044 4.32816987397837e-09 454749.8290356 -610230.74899327;-0.0004 4.76443685547352e-09 463899.795656877 -603304.214546686;-0.00036 5.19962044511449e-09 472944.275465123 -596240.493924388;-0.00032 5.63362168590585e-09 481881.211823625 -589041.193355531;-0.00028 6.06634188970812e-09 490708.572550126 -581707.949898979;-0.00024 6.49768265967858e-09 499424.350378919 -574242.431071057;-0.0002 6.92754591264585e-09 508026.563417289 -566646.334466364;-0.00016 7.3558339014132e-09 516513.255596171 -558921.387371763;-0.00012 7.78244923698538e-09 524882.497114952 -551069.346373608;-8e-05 8.20729491071406e-09 533132.384880283 -543091.996958306;-4e-05 8.63027431635673e-09 541261.04293883 -534991.153106322]  x2=[-0.00124 -1.45754569638302e-08 124927.718475594 -772311.093224702;-0.0012 -1.3323989710404e-08 136559.222590638 -770339.54939026;-0.00116 -1.20694926966187e-08 148159.674316101 -768192.836985412;-0.00112 -1.08122511842772e-08 159726.435809299 -765871.444154046;-0.00108 -9.55255105925721e-09 171256.876888417 -763375.898760874;-0.00104 -8.29067876650404e-09 182748.375630586 -760706.768271397;-0.001 -7.02692124489515e-09 194198.318968092 -757864.65962287;-0.00096 -5.76156586199275e-09 205604.103282559 -754850.219086292;-0.00092 -4.49490034869897e-09 216963.134996994 -751664.132119445;-0.00088 -3.22721273382825e-09 228272.831165542 -748307.123211029;-0.00084 -1.95879127861217e-09 239530.620060823 -744779.955715921;-0.0008 -6.89924411151219e-10 250733.941758726 -741083.431681592;-0.00076 5.7909933917117e-10 261880.248720511 -737218.39166573;-0.00072 1.84799140729777e-09 272967.006372097 -733185.714545103;-0.00068 3.11646325811475e-09 283991.6936804 -728986.317315714;-0.00064 4.38422645206207e-09 294951.8037266 -724621.154884277;-0.0006 5.65099271072215e-09 305844.844276189 -720091.219851086;-0.00056 6.91647398237189e-09 316668.338345683 -715397.542284303;-0.00052 8.18038250748318e-09 327419.824765869 -710541.18948573;-0.00048 9.44243088415688e-09 338096.858741452 -705523.265748115;-0.00044 1.07023321334756e-08 348697.012406979 -700344.912104042;-0.0004 1.19597997647601e-08 359217.875378921 -695007.306066474;-0.00036 1.3214547840715e-08 369657.055303764 -689511.661360994;-0.00032 1.44662910424484e-08 380012.178402018 -683859.227649815;-0.00028 1.57147447343507e-08 390280.890007988 -678051.29024762;-0.00024 1.69596250288186e-08 400460.85510521 -672089.169829288;-0.0002 1.82006488508085e-08 410549.758857408 -665974.222129588;-0.00016 1.94375340022055e-08 420545.307134873 -659707.837634891;-0.00012 2.06699992259925e-08 430445.227036123 -653291.441266995;-8e-05 2.1897764270206e-08 440247.267404747 -646726.4920591;-4e-05 2.31205499516627e-08 449949.199341294 -640014.482824043]  x3=[-0.00124 -5.03388116047608e-10 -674.173767516043 -3326.18343649101;-0.0012 -5.01425518902876e-10 -623.941715224432 -3335.97193728453;-0.00116 -4.99348901919255e-10 -573.567783967424 -3345.00186682771;-0.00112 -4.97158737301538e-10 -523.063428342579 -3353.27117179244;-0.00108 -4.94855523074274e-10 -472.440132604836 -3360.77797181009;-0.00104 -4.92439782968515e-10 -421.709408055089 -3367.52055989906;-0.001 -4.89912066302729e-10 -370.882790422617 -3373.49740285296;-0.00096 -4.87272947857887e-10 -319.97183724196 -3378.70714158927;-0.00092 -4.84523027746765e-10 -268.988125224835 -3383.1485914583;-0.00088 -4.81662931277483e-10 -217.943247627687 -3386.82074251267;-0.00084 -4.78693308811312e-10 -166.848811615492 -3389.72275973689;-0.0008 -4.75614835614792e-10 -115.716435622378 -3391.85398323726;-0.00076 -4.72428211706182e-10 -64.5577467096992 -3393.21392839196;-0.00072 -4.69134161696277e-10 -13.3843779221413 -3393.80228596117;-0.00068 -4.65733434623642e-10 37.7920343575341 -3393.61892215745;-0.00064 -4.62226803784289e-10 88.9598530545012 -3392.66387867616;-0.0006 -4.58615066555829e-10 140.107443048041 -3390.93737268594;-0.00056 -4.54899044216162e-10 191.223173817267 -3388.43979677938;-0.00052 -4.51079581756723e-10 242.295422085805 -3385.17171888369;-0.00048 -4.47157547690337e-10 293.312574464827 -3381.1338821316;-0.00044 -4.43133833853729e-10 344.263030093836 -3376.32720469237;-0.0004 -4.39009355204725e-10 395.1352032786 -3370.752779563;-0.00036 -4.34785049614204e-10 445.917526125639 -3364.41187431969;-0.00032 -4.30461877652827e-10 496.598451172666 -3357.30593082961;-0.00028 -4.26040822372616e-10 547.166454014379 -3349.43656492304;-0.00024 -4.21522889083418e-10 597.610035923011 -3340.80556602591;-0.0002 -4.16909105124301e-10 647.917726463045 -3331.41489675295;-0.00016 -4.1220051962995e-10 698.078086099484 -3321.26669246136;-0.00012 -4.073982032921e-10 748.079708799115 -3310.3632607653;-8e-05 -4.02503248116075e-10 797.911224624128 -3298.70708101109;-4e-05 -3.97516767172468e-10 847.561302317556 -3286.3008037135]  x4=[-0.00124 3.30056474968153e-10 2485.54609255125 -13653.4102513513;-0.0012 3.34191422386142e-10 2691.14422271432 -13614.3788533336;-0.00116 3.38250377556625e-10 2896.13040988858 -13572.2516629701;-0.00112 3.42232417508198e-10 3100.4580419828 -13527.0382596205;-0.00108 3.46136636759317e-10 3304.08065665549 -13478.7489244229;-0.00104 3.49962147524191e-10 3506.95195188002 -13427.3946379557;-0.001 3.53708079914664e-10 3709.02579647337 -13372.9870777407;-0.00096 3.57373582138013e-10 3910.25624058587 -13315.5386155879;-0.00092 3.60957820690642e-10 4110.59752614988 -13255.0623147823;-0.00088 3.64459980547613e-10 4310.00409728473 -13191.5719271131;-0.00084 3.67879265347977e-10 4508.43061065574 -13125.081889747;-0.0008 3.71214897575857e-10 4705.83194578495 -13055.607321945;-0.00076 3.74466118737249e-10 4902.16321531104 -12983.1640216248;-0.00072 3.77632189532498e-10 5097.37977519643 -12907.768461768;-0.00068 3.80712390024409e-10 5291.43723487888 -12829.437786675;-0.00064 3.83706019801952e-10 5484.29146736552 -12748.1898080656;-0.0006 3.86612398139532e-10 5675.89861926699 -12664.0430010295;-0.00056 3.89430864151778e-10 5866.21512076932 -12577.0164998251;-0.00052 3.92160776943825e-10 6055.19769554126 -12487.1300935282;-0.00048 3.94801515757045e-10 6242.80337057504 -12394.4042215324;-0.00044 3.97352480110206e-10 6428.98948595799 -12298.8599689015;-0.0004 3.99813089936011e-10 6613.71370457308 -12200.5190615745;-0.00036 4.02182785713006e-10 6796.93402172599 -12099.4038614256;-0.00032 4.04461028592807e-10 6978.60877469662 -11995.5373611795;-0.00028 4.06647300522629e-10 7158.69665221284 -11888.9431791826;-0.00024 4.08741104363089e-10 7337.15670384432 -11779.6455540326;-0.0002 4.1074196400125e-10 7513.94834931429 -11667.6693390669;-0.00016 4.12649424458885e-10 7689.03138772716 -11553.0399967113;-0.00012 4.14463051995935e-10 7862.36600670984 -11435.7835926896;-8e-05 4.16182434209139e-10 8033.91279146476 -11315.9267900969;-4e-05 4.17807180125808e-10 8203.6327337324 -11193.4968433365]  x5=0.00123288061605072  V1=ones(3,3)  V2=ones(3,3)  I1=ones(3,3)  I2=ones(3,3)  nHarmo=1  Measurements=None
      settings: AttributesFormatString=\n  SourceProductName=Simscape Power Systems
  LMO7 : powerlib/Measurements/Three-Phase V-I Measurement  VoltageMeasurement=no  SetLabelV=on  LabelV=Vabc_LMO7  Vpu=on  VpuLL=off  CurrentMeasurement=no  SetLabelI=off  LabelI=A1  Ipu=off  Pbase=100e6  Vbase=735e3  OutputType=Magnitude  PhasorSimulation=off  PSBequivalent=0
  LVD 990 Mvar : powerlib/Elements/Three-Phase Series RLC Load  LConnTagsString=A|B|C  Configuration=Y (grounded)  NominalVoltage=735e3  Vabc=[1e3 1e3 1e3]  Vabcp=[1e3 1e3 1e3]  NominalFrequency=60  UnbalancedPower=off  ActivePower=3300000  InductivePower=990e6  CapacitivePower=0  Pabc=[10e3 9e3 11e3]  QLabc=[100 90 110]  QCabc=[100 90 110]  Pabcp=[10e3 9e3 11e3]  QLabcp=[100 90 110]  QCabcp=[100 90 110]  Measurements=None  LoadType=constant Z
  LVD-MTL 3*260km : powerlib/Elements/Distributed Parameters Line  Phases=3  Frequency=60  Resistance="[0.01273  0.3864]/3"  Inductance="[0.9337e-3  4.1264e-3]/3"  Capacitance=[12.74e-9 7.751e-9]*3  Length=260  x1=[-0.00148 -6.94851673709031e-08 -108995.715576429 -808302.335136461;-0.00144 -6.54526014771003e-08 -96794.894585085 -809854.045778418;-0.0014 -6.14051522261608e-08 -84572.0632694361 -811221.60259425;-0.00136 -5.73437399731405e-08 -72330.0009959184 -812404.694613328;-0.00132 -5.32692882481618e-08 -60071.4915039214 -813403.052810732;-0.00128 -4.91827235464101e-08 -47799.3222727909 -814216.450168415;-0.00124 -4.50849751174578e-08 -35516.2838879795 -814844.701726833;-0.0012 -4.097697475396e-08 -23225.1694064912 -815287.664627001;-0.00116 -3.68596565797736e-08 -10928.7737217654 -815545.238142973;-0.00112 -3.2733956837545e-08 1370.10707185916 -815617.363704755;-0.00108 -2.86008136758172e-08 13668.6763149508 -815504.024911614;-0.00104 -2.44611669357025e-08 25964.1374189222 -815205.247535816;-0.001 -2.03159579371706e-08 38253.6945019497 -814721.099516759;-0.00096 -1.61661292650013e-08 50534.5530247331 -814051.690945527;-0.00092 -1.20126245544478e-08 62803.9204259501 -813197.174039857;-0.00088 -7.85638827666311e-09 75059.0067572604 -812157.743109524;-0.00084 -3.69836552393491e-09 87297.0253177152 -810933.634512158;-0.0008 4.60498205220074e-10 99515.1932874303 -809525.126599498;-0.00076 4.61925722105438e-09 111710.732360374 -807932.539654096;-0.00072 8.77696585763139e-09 123880.869376132 -806156.235816491;-0.00068 1.29326786878617e-08 136022.836950497 -804196.619002856;-0.00064 1.70854507384851e-08 148133.87410475 -802054.134813157;-0.0006 2.12343377049491e-08 160211.226893483 -799729.270429821;-0.00056 2.53783961661362e-08 172252.149030824 -797222.554506961;-0.00052 2.95166837988891e-08 184253.902514915 -794534.55705016;-0.00048 3.36482595922872e-08 196213.758250512 -791665.88928686;-0.00044 3.77721840616242e-08 208128.996669558 -788617.203527373;-0.0004 4.1887519462039e-08 219996.908349589 -785389.193016548;-0.00036 4.59933300017508e-08 231814.794629834 -781982.59177614;-0.00032 5.00886820548497e-08 243579.968224866 -778398.174437892;-0.00028 5.41726443735958e-08 255289.753835668 -774636.756067397;-0.00024 5.82442883001763e-08 266941.488757972 -770699.191978755;-0.0002 6.23026879778747e-08 278532.523487739 -766586.377540084;-0.00016 6.63469205616024e-08 290060.222323626 -762299.247969919;-0.00012 7.03760664277459e-08 301521.96396633 -757838.778124556;-8e-05 7.43892093832811e-08 312915.142114643 -753205.982276369;-4e-05 7.83854368741077e-08 324237.166058104 -748401.913883185]  x2=[-0.00148 -9.09013898329145e-08 -330739.237201115 -730967.879631096;-0.00144 -8.48734926170629e-08 -319679.329182502 -735872.056438699;-0.0014 -7.88262959009079e-08 -308546.728841231 -740608.902286558;-0.00136 -7.27611747648342e-08 -297343.967634614 -745177.340056776;-0.00132 -6.66795083650845e-08 -286073.592973943 -749576.330926;-0.00128 -6.05826796201523e-08 -274738.167645223 -753804.874601644;-0.00124 -5.44720748963172e-08 -263340.269226422 -757862.009549339;-0.0012 -4.83490836923978e-08 -251882.489501348 -761746.813211586;-0.00116 -4.22150983237915e-08 -240367.433870303 -765458.402217534;-0.00112 -3.60715136058739e-08 -228797.720757637 -768995.932583849;-0.00108 -2.99197265368299e-08 -217175.981016339 -772358.599906634;-0.00104 -2.3761135979988e-08 -205504.857329803 -775545.639544336;-0.001 -1.75971423457316e-08 -193787.003610908 -778556.326791627;-0.00096 -1.14291472730571e-08 -182025.084398541 -781389.97704419;-0.00092 -5.25855331085351e-09 -170221.774251699 -784045.945954392;-0.00088 9.13236401025173e-10 -158379.757141322 -786523.629577809;-0.00084 7.08481845082168e-09 -146501.725839979 -788822.464510551;-0.0008 1.32547894739993e-08 -134590.381309558 -790941.928017378;-0.00076 1.94217464723551e-08 -122648.432087085 -792881.538150567;-0.00072 2.5584287133049e-08 -110678.593668831 -794640.8538595;-0.00068 3.17410101474783e-08 -98683.5878928279 -796219.475090956;-0.00064 3.78905155299229e-08 -86666.1423199488 -797617.04288008;-0.0006 4.40314049358899e-08 -74628.9896136833 -798833.23943201;-0.00056 5.01622819800852e-08 -62574.8669187526 -799867.788194138;-0.00052 5.62817525539393e-08 -50506.5152387072 -800720.453918996;-0.00048 6.23884251426157e-08 -38426.6788126462 -801391.042717752;-0.00044 6.84809111414296e-08 -26338.1044912007 -801879.402104296;-0.0004 7.45578251716042e-08 -14243.5411119241 -802185.421029915;-0.00036 8.06177853952941e-08 -2145.73887422974 -802309.029908544;-0.00032 8.66594138298032e-08 9952.55128598059 -802250.200632591;-0.00028 9.26813366609264e-08 22048.5783218556 -802008.946579325;-0.00024 9.86821845553427e-08 34139.5917011591 -801585.322607837;-0.0002 1.0466059297199e-07 46222.8420317171 -800979.425046565;-0.00016 1.1061520247235e-07 58295.5816866058 -800191.391671391;-0.00012 1.16544659029573e-07 70355.0654289387 -799221.401674307;-8e-05 1.2244761433637e-07 82398.5510361093 -798069.675622674;-4e-05 1.28322726111611e-07 94423.2999233492 -796736.475409064]  x3=[-0.00148 -1.49708929615689e-09 -410.698657158697 -1224.82685921688;-0.00144 -1.48221799979119e-09 -392.183267372481 -1230.88095063406;-0.0014 -1.46700965983445e-09 -373.578698493308 -1236.65515033773;-0.00136 -1.45146773453201e-09 -354.889181039703 -1242.14814532468;-0.00132 -1.43559575798367e-09 -336.118964846764 -1247.3586865352;-0.00128 -1.41939733934001e-09 -317.272318099785 -1252.28558913717;-0.00124 -1.40287616198175e-09 -298.35352636371 -1256.92773279542;-0.0012 -1.38603598268213e-09 -279.366891608631 -1261.28406192652;-0.00116 -1.36888063075273e-09 -260.316731231558 -1265.35358593879;-0.00112 -1.35141400717261e-09 -241.207377074679 -1269.13537945755;-0.00108 -1.33364008370136e-09 -222.043174440337 -1272.62858253559;-0.00104 -1.3155629019759e-09 -202.828481102946 -1275.83240084864;-0.001 -1.29718657259146e-09 -183.56766631807 -1278.74610587605;-0.00096 -1.27851527416688e-09 -164.265109828894 -1281.36903506641;-0.00092 -1.25955325239439e-09 -144.925200870305 -1283.70059198826;-0.00088 -1.24030481907424e-09 -125.552337170819 -1285.74024646565;-0.00084 -1.22077435113416e-09 -106.150923952579 -1287.48753469875;-0.0008 -1.20096628963414e-09 -86.7253729296374 -1288.94205936928;-0.00076 -1.18088513875655e-09 -67.2801013047798 -1290.10348973087;-0.00072 -1.16053546478193e-09 -47.8195307650844 -1290.97156168427;-0.00068 -1.13992189505065e-09 -28.3480864764711 -1291.54607783742;-0.00064 -1.1190491169107e-09 -8.87019607745645 -1291.82690755028;-0.0006 -1.09792187665184e-09 10.6097113276528 -1291.8139869646;-0.00056 -1.0765449784263e-09 30.0872061759004 -1291.50731901842;-0.00052 -1.05492328315639e-09 49.5578594529246 -1290.90697344538;-0.00048 -1.03306170742917e-09 69.0172437000781 -1290.01308675888;-0.00044 -1.01096522237842e-09 88.4609340211935 -1288.82586222105;-0.0004 -9.88638852554291e-10 107.884509088767 -1287.34556979652;-0.00036 -9.66087674780753e-10 127.28355214933 -1285.57254609101;-0.00032 -9.43316817001155e-10 146.653652027781 -1283.50719427482;-0.00028 -9.20331457112188e-10 165.990404130448 -1281.14998399115;-0.00024 -8.97136821786475e-10 185.289411446656 -1278.50145124929;-0.0002 -8.73738185284066e-10 204.546285548569 -1275.56219830274;-0.00016 -8.50140868253121e-10 223.756647589081 -1272.33289351228;-0.00012 -8.26350236520037e-10 242.916129297525 -1268.81427119396;-8e-05 -8.0237169986931e-10 262.020373972987 -1265.00713145216;-4e-05 -7.78210710813391e-10 281.065037474975 -1260.91233999763]  x4=[-0.00148 1.74599064204203e-10 -7310.64461779518 -14849.0635067736;-0.00144 1.94368996529732e-10 -7085.90295274095 -14957.613751333;-0.0014 2.14094731021616e-10 -6859.55001446148 -15062.7627635143;-0.00136 2.33771782217941e-10 -6631.63727366297 -15164.4866333388;-0.00132 2.53395675726951e-10 -6402.21655573723 -15262.762229676;-0.00128 2.72961949244492e-10 -6171.34002897708 -15357.5672055025;-0.00124 2.92466153568699e-10 -5939.06019271372 -15448.8800029846;-0.0012 3.11903853611705e-10 -5705.4298653788 -15536.6798583794;-0.00116 3.31270629408143e-10 -5470.50217249403 -15620.946806757;-0.00112 3.50562077120211e-10 -5234.33053459083 -15701.6616865401;-0.00108 3.6977381003906e-10 -4996.96865506301 -15778.8061438611;-0.00104 3.88901459582299e-10 -4758.47050795505 -15852.3626367356;-0.001 4.07940676287373e-10 -4518.89032568889 -15922.3144390514;-0.00096 4.2688713080059e-10 -4278.28258673191 -15988.645644372;-0.00092 4.4573651486158e-10 -4036.70200320905 -16051.3411695532;-0.00088 4.64484542282959e-10 -3794.2035084617 -16110.3867581734;-0.00084 4.83126949924967e-10 -3550.84224455634 -16165.7689837748;-0.0008 5.01659498664872e-10 -3306.67354974572 -16217.4752529169;-0.00076 5.20077974360907e-10 -3061.75294588543 -16265.4938080401;-0.00072 5.38378188810534e-10 -2816.13612580868 -16309.813730139;-0.00068 5.56555980702801e-10 -2569.87894066225 -16350.4249412455;-0.00064 5.74607216564591e-10 -2323.0373872064 -16387.3182067205;-0.0006 5.92527791700536e-10 -2075.66759508172 -16420.4851373534;-0.00056 6.1031363112639e-10 -1827.82581404571 -16449.9181912703;-0.00052 6.27960690495646e-10 -1579.56840118209 -16475.6106756486;-0.00048 6.45464957019186e-10 -1330.95180808566 -16497.5567482389;-0.00044 6.62822450377753e-10 -1082.03256802571 -16515.7514186934;-0.0004 6.80029223627041e-10 -832.867283090838 -16530.1905497012;-0.00036 6.97081364095198e-10 -583.512611318136 -16540.8708579282;-0.00032 7.13974994272534e-10 -334.025253809618 -16547.7899147645;-0.00028 7.30706272693231e-10 -84.4619418388952 -16550.9461468763;-0.00024 7.47271394808859e-10 165.120576049033 -16550.3388365636;-0.0002 7.63666593853503e-10 414.665546941907 -16545.9681219235;-0.00016 7.79888141700284e-10 664.11622646533 -16537.8349968187;-0.00012 7.95932349709111e-10 913.415891685949 -16525.941310652;-8e-05 8.11795569565443e-10 1162.50785400976 -16510.2897679448;-4e-05 8.27474194109882e-10 1411.33547207261 -16490.8839277231]  x5=0.00147040807418893  V1=ones(3,3)  V2=ones(3,3)  I1=ones(3,3)  I2=ones(3,3)  nHarmo=1  Measurements=None
      settings: AttributesFormatString=\n  SourceProductName=Simscape Power Systems
  LVD7 : powerlib/Measurements/Three-Phase V-I Measurement  VoltageMeasurement=no  SetLabelV=on  LabelV=Vabc_LVD7  Vpu=on  VpuLL=off  CurrentMeasurement=no  SetLabelI=off  LabelI=A1  Ipu=off  Pbase=100e6  Vbase=735e3  OutputType=Magnitude  PhasorSimulation=off  PSBequivalent=0
  Load Flow Bus1 : powerlib/Measurements/Load Flow Bus  LConnTagsString=a  Phases=single  Connectors=on one side  ID=LG31_13.8  Vbase=13.8e3  Vref=1  Vangle=0  VLF=1  VLFb=1  VLFc=1  angleLF=-1.034  angleLFb=0  angleLFc=0
      settings: AttributesFormatString=%<ID>\n%<Vbase>V\n%<VLF>pu\n%<angleLF>deg.  SourceProductName=Simscape Power Systems
  Load Flow Bus10 : powerlib/Measurements/Load Flow Bus  LConnTagsString=a  Phases=single  Connectors=on one side  ID=LVD7  Vbase=735e3  Vref=1  Vangle=0  VLF=1.12  VLFb=1  VLFc=1  angleLF=-11.83  angleLFb=0  angleLFc=0
      settings: AttributesFormatString=%<ID>\n%<Vbase>V\n%<VLF>pu\n%<angleLF>deg.  SourceProductName=Simscape Power Systems
  Load Flow Bus11 : powerlib/Measurements/Load Flow Bus  LConnTagsString=a  Phases=single  Connectors=on one side  ID=CHM7  Vbase=735e3  Vref=1  Vangle=0  VLF=1.103  VLFb=1  VLFc=1  angleLF=-4.5  angleLFb=0  angleLFc=0
      settings: AttributesFormatString=%<ID>\n%<Vbase>V\n%<VLF>pu\n%<angleLF>deg.  SourceProductName=Simscape Power Systems
  Load Flow Bus12 : powerlib/Measurements/Load Flow Bus  LConnTagsString=a  Phases=single  Connectors=on one side  ID=LG47  Vbase=735e3  Vref=1  Vangle=0  VLF=1.016  VLFb=1  VLFc=1  angleLF=19.5  angleLFb=0  angleLFc=0
      settings: AttributesFormatString=%<ID>\n%<Vbase>V\n%<VLF>pu\n%<angleLF>deg.  SourceProductName=Simscape Power Systems
  Load Flow Bus2 : powerlib/Measurements/Load Flow Bus  LConnTagsString=a  Phases=single  Connectors=on one side  ID=LG3_13.8  Vbase=13.8e3  Vref=1  Vangle=0  VLF=1  VLFb=1  VLFc=1  angleLF=-1.597  angleLFb=0  angleLFc=0
      settings: AttributesFormatString=%<ID>\n%<Vbase>V\n%<VLF>pu\n%<angleLF>deg.  SourceProductName=Simscape Power Systems
  Load Flow Bus3 : powerlib/Measurements/Load Flow Bus  LConnTagsString=a  Phases=single  Connectors=on one side  ID=LG4_13.8  Vbase=13.8e3  Vref=1  Vangle=0  VLF=1  VLFb=1  VLFc=1  angleLF=-4.546  angleLFb=0  angleLFc=0
      settings: AttributesFormatString=%<ID>\n%<Vbase>V\n%<VLF>pu\n%<angleLF>deg.  SourceProductName=Simscape Power Systems
  Load Flow Bus4 : powerlib/Measurements/Load Flow Bus  LConnTagsString=a  Phases=single  Connectors=on one side  ID=LG2_13.8  Vbase=13.8e3  Vref=1  Vangle=0  VLF=1  VLFb=1  VLFc=1  angleLF=0  angleLFb=0  angleLFc=0
      settings: AttributesFormatString=%<ID>\n%<Vbase>V\n%<VLF>pu\n%<angleLF>deg.  SourceProductName=Simscape Power Systems
  Load Flow Bus5 : powerlib/Measurements/Load Flow Bus  LConnTagsString=a  Phases=single  Connectors=on one side  ID=LG27  Vbase=735e3  Vref=1  Vangle=0  VLF=1.009  VLFb=1  VLFc=1  angleLF=23.08  angleLFb=0  angleLFc=0
      settings: AttributesFormatString=%<ID>\n%<Vbase>V\n%<VLF>pu\n%<angleLF>deg.  SourceProductName=Simscape Power Systems
  Load Flow Bus6 : powerlib/Measurements/Load Flow Bus  LConnTagsString=a  Phases=single  Connectors=on one side  ID=LG37  Vbase=735e3  Vref=1  Vangle=0  VLF=1.002  VLFb=1  VLFc=1  angleLF=23.14  angleLFb=0  angleLFc=0
      settings: AttributesFormatString=%<ID>\n%<Vbase>V\n%<VLF>pu\n%<angleLF>deg.  SourceProductName=Simscape Power Systems
  Load Flow Bus7 : powerlib/Measurements/Load Flow Bus  LConnTagsString=a  Phases=single  Connectors=on one side  ID=LMO7  Vbase=735e3  Vref=1  Vangle=0  VLF=1.035  VLFb=1  VLFc=1  angleLF=16.2  angleLFb=0  angleLFc=0
      settings: AttributesFormatString=%<ID>\n%<Vbase>V\n%<VLF>pu\n%<angleLF>deg.  SourceProductName=Simscape Power Systems
  Load Flow Bus8 : powerlib/Measurements/Load Flow Bus  LConnTagsString=a  Phases=single  Connectors=on one side  ID=NEM_ALB7  Vbase=735e3  Vref=1  Vangle=0  VLF=1.063  VLFb=1  VLFc=1  angleLF=8.044  angleLFb=0  angleLFc=0
      settings: AttributesFormatString=%<ID>\n%<Vbase>V\n%<VLF>pu\n%<angleLF>deg.  SourceProductName=Simscape Power Systems
  Load Flow Bus9 : powerlib/Measurements/Load Flow Bus  LConnTagsString=a  Phases=single  Connectors=on one side  ID=ABI_CHB7  Vbase=735e3  Vref=1  Vangle=0  VLF=1.096  VLFb=1  VLFc=1  angleLF=-0.4779  angleLFb=0  angleLFc=0
      settings: AttributesFormatString=%<ID>\n%<Vbase>V\n%<VLF>pu\n%<angleLF>deg.  SourceProductName=Simscape Power Systems
  NEM-ABI 6*236 : powerlib/Elements/Distributed Parameters Line  Phases=3  Frequency=60  Resistance="[0.01273  0.3864]/6"  Inductance="[0.9337e-3  4.1264e-3]/6"  Capacitance=[12.74e-9 7.751e-9]*6  Length=236  x1=[-0.00136 -1.8430221216744e-08 0 0;-0.00132 -1.72222918042574e-08 0 0;-0.00128 -1.60104461911333e-08 0 0;-0.00124 -1.47949599406135e-08 0 0;-0.0012 -1.35761094437895e-08 0 0;-0.00116 -1.23541718567534e-08 0 0;-0.00112 -1.11294250375749e-08 0 0;-0.00108 -9.90214748311893e-09 0 0;-0.00104 -8.67261826571778e-09 0 0;-0.001 -7.44111696971248e-09 0 0;-0.00096 -6.20792362787773e-09 0 0;-0.00092 -4.97331865774484e-09 0 0;-0.00088 -3.73758279783727e-09 0 0;-0.00084 -2.500997043833e-09 265985.505991479 -734731.96796445;-0.0008 -1.26384258466865e-09 277034.305223583 -730637.672527718;-0.00076 -2.64007385994577e-11 288020.109243722 -726377.236385003;-0.00072 1.21104711077002e-09 298940.419974798 -721951.628322745;-0.00068 2.44821957847014e-09 309792.754232325 -717361.854686053;-0.00064 3.68483534215066e-09 320574.644289078 -712608.95914987;-0.0006 4.92061320605104e-09 331283.638436237 -707694.022481654;-0.00056 6.15527216494192e-09 341917.301540885 -702618.162295619;-0.00052 7.38853146802331e-09 352473.215599732 -697382.532798599;-0.00048 8.62011068276484e-09 362948.98028895 -691988.324527591;-0.00044 9.84972975867379e-09 373342.21350999 -686436.764079039;-0.0004 1.10771090909761e-08 383650.551931244 -680729.113829914;-0.00036 1.2301969584196e-08 393871.651525449 -674866.671650662;-0.00032 1.35240327156201e-08 404003.188102703 -668850.770610079;-0.00028 1.4743020598631e-08 414042.857838957 -662682.778672183;-0.00024 1.59586560458961e-08 423988.377799892 -656364.098385149;-0.0002 1.7170662632398e-08 433837.486460035 -649896.166562386;-0.00016 1.83787647582908e-08 443587.944217013 -643280.453955812;-0.00012 1.95826877115693e-08 453237.533900815 -636518.464921423;-8e-05 2.0782157730536e-08 462784.061277962 -629611.737077212;-4e-05 2.19769020660526e-08 472225.355550454 -622561.84095353]  x2=[-0.00136 -2.7519361540281e-08 0 0;-0.00132 -2.54039924013673e-08 0 0;-0.00128 -2.32828466136563e-08 0 0;-0.00124 -2.1156406507408e-08 0 0;-0.0012 -1.90251556167651e-08 0 0;-0.00116 -1.68895785698008e-08 0 0;-0.00112 -1.47501609783193e-08 0 0;-0.00108 -1.26073893274313e-08 0 0;-0.00104 -1.04617508649317e-08 0 0;-0.001 -8.31373349050372e-09 0 0;-0.00096 -6.16382564477462e-09 0 0;-0.00092 -4.01251619824843e-09 0 0;-0.00088 -1.86029434014124e-09 0 0;-0.00084 2.92350532856405e-10 110748.824006098 -800359.440643582;-0.0008 2.444928927864e-09 122804.875797586 -798598.502540886;-0.00076 4.59695136711756e-09 134833.002819341 -796655.970025532;-0.00072 6.74792849927266e-09 146830.469979006 -794532.284812663;-0.00068 8.89737121067869e-09 158794.549156009 -792227.929809982;-0.00064 1.10447907365991e-08 170722.51982192 -789743.429007945;-0.0006 1.31896987723522e-08 182611.669659072 -787079.347360609;-0.00056 1.53316075843476e-08 194459.295177319 -784236.290657167;-0.00052 1.74700301209924e-08 206262.702328789 -781214.905384194;-0.00048 1.96044801234429e-08 218019.207120483 -778015.878578648;-0.00044 2.17344722361751e-08 229726.136224595 -774639.937671636;-0.0004 2.38595221173509e-08 241380.827586404 -771087.850323008;-0.00036 2.5979146548953e-08 252980.631029599 -767360.424246795;-0.00032 2.80928635466645e-08 264522.90885891 -763458.507027542;-0.00028 3.0200192469468e-08 276005.036459894 -759382.985927578;-0.00024 3.23006541289394e-08 287424.402895754 -755134.787685253;-0.0002 3.43937708982107e-08 298778.411501038 -750714.878304214;-0.00016 3.64790668205791e-08 310064.480472102 -746124.262833738;-0.00012 3.85560677177345e-08 321280.043454189 -741363.985140195;-8e-05 4.06243012975844e-08 332422.550124995 -736435.127669681;-4e-05 4.26832972616481e-08 343489.466774593 -731338.811201882]  x3=[-0.00136 -1.24320141770731e-09 0 0;-0.00132 -1.23343965856954e-09 0 0;-0.00128 -1.22339742589014e-09 0 0;-0.00124 -1.21307700318623e-09 0 0;-0.0012 -1.20248073723292e-09 0 0;-0.00116 -1.19161103752971e-09 0 0;-0.00112 -1.18047037575259e-09 0 0;-0.00108 -1.16906128519196e-09 0 0;-0.00104 -1.15738636017664e-09 0 0;-0.001 -1.14544825548389e-09 0 0;-0.00096 -1.13324968573576e-09 0 0;-0.00092 -1.12079342478183e-09 0 0;-0.00088 -1.10808230506841e-09 0 0;-0.00084 -1.09511921699452e-09 -1841.98186161868 -5911.45634354616;-0.0008 -1.08190710825459e-09 -1752.63423005462 -5938.56084166786;-0.00076 -1.0684489831682e-09 -1662.88806458073 -5964.31496226613;-0.00072 -1.05474790199696e-09 -1572.76377270108 -5988.71284907605;-0.00068 -1.04080698024857e-09 -1482.28184790246 -6011.74895422855;-0.00064 -1.0266293879684e-09 -1391.46286499428 -6033.41803951197;-0.0006 -1.01221834901868e-09 -1300.32747543007 -6053.71517756319;-0.00056 -9.97577140345395e-10 -1208.89640261149 -6072.63575298805;-0.00052 -9.82709091233134e-10 -1117.19043717604 -6090.17546341086;-0.00048 -9.67617582548049e-10 -1025.23043226941 -6106.33032045272;-0.00044 -9.52306045969071e-10 -933.037298803691 -6121.09665063846;-0.0004 -9.36777963207578e-10 -840.632000702398 -6134.47109623194;-0.00036 -9.2103686521568e-10 -748.035550133446 -6146.45061599956;-0.00032 -9.05086331383315e-10 -655.269002731178 -6157.03248590183;-0.00028 -8.88929988724326e-10 -562.353452808489 -6166.2142997128;-0.00024 -8.72571511051707e-10 -469.31002856016 -6173.99396956718;-0.0002 -8.56014618142212e-10 -376.159887258494 -6180.36972643513;-0.00016 -8.39263074890506e-10 -282.92421044233 -6185.34012052454;-0.00012 -8.22320690453066e-10 -189.624199100546 -6188.90402161064;-8e-05 -8.0519131738201e-10 -96.281068851136 -6191.06061929305;-4e-05 -7.87878850749054e-10 -2.91604511696186 -6191.80942318008]  x4=[-0.00136 4.57341603079404e-10 0 0;-0.00132 4.71147144440377e-10 0 0;-0.00128 4.84845551003705e-10 0 0;-0.00124 4.98433707869864e-10 0 0;-0.0012 5.11908525209163e-10 0 0;-0.00116 5.2526693896434e-10 0 0;-0.00112 5.38505911547306e-10 0 0;-0.00108 5.51622432529864e-10 0 0;-0.00104 5.64613519328253e-10 0 0;-0.001 5.77476217881367e-10 0 0;-0.00096 5.90207603322477e-10 0 0;-0.00092 6.02804780644326e-10 0 0;-0.00088 6.15264885357423e-10 0 0;-0.00084 6.27585084141408e-10 4889.70242731462 -29110.9932620945;-0.0008 6.39762575489322e-10 5328.11314559195 -29033.9525972077;-0.00076 6.51794590344648e-10 5765.31229688766 -28950.3098618784;-0.00072 6.63678392730966e-10 6201.20046588499 -28860.0840757433;-0.00068 6.75411280374097e-10 6635.67853537326 -28763.2957553682;-0.00064 6.86990585316569e-10 7068.64770878624 -28659.9669095825;-0.0006 6.98413674524294e-10 7500.00953266766 -28550.1210344745;-0.00056 7.09677950485296e-10 7929.66591905868 -28433.783108049;-0.00052 7.20780851800359e-10 8357.51916780223 -28310.9795845473;-0.00048 7.31719853765472e-10 8783.4719887592 -28181.7383884315;-0.00044 7.42492468945923e-10 9207.42752393136 -28046.0889080352;-0.0004 7.53096247741917e-10 9629.28936948606 -27904.0619888803;-0.00036 7.635287789456e-10 10048.9615976776 -27755.6899266636;-0.00032 7.73787690289343e-10 10466.3487786604 -27601.0064599124;-0.00028 7.83870648985175e-10 10881.3560021888 -27440.0467623131;-0.00024 7.9377536225524e-10 11293.8888991992 -27272.847434713;-0.0002 8.03499577853155e-10 11703.8536632682 -27099.4464967973;-0.00016 8.13041084576152e-10 12111.157071944 -26919.8833784439;-0.00012 8.22397712767884e-10 12515.7065079437 -26734.1989107573;-8e-05 8.31567334811788e-10 12917.4099802144 -26542.4353167845;-4e-05 8.40547865614888e-10 13316.1761448506 -26344.6362019127]  x5=0.00133467809810995  V1=ones(3,3)  V2=ones(3,3)  I1=ones(3,3)  I2=ones(3,3)  nHarmo=1  Measurements=None
      settings: AttributesFormatString=\n  SourceProductName=Simscape Power Systems
  NEM-ALB 1980 Mvar : powerlib/Elements/Three-Phase Series RLC Load  LConnTagsString=A|B|C  Configuration=Y (grounded)  NominalVoltage=735e3  Vabc=[1e3 1e3 1e3]  Vabcp=[1e3 1e3 1e3]  NominalFrequency=60  UnbalancedPower=off  ActivePower=6600000  InductivePower=1980e6  CapacitivePower=0  Pabc=[10e3 9e3 11e3]  QLabc=[100 90 110]  QCabc=[100 90 110]  Pabcp=[10e3 9e3 11e3]  QLabcp=[100 90 110]  QCabcp=[100 90 110]  Measurements=None  LoadType=constant Z
  NEM-ALB7 : powerlib/Measurements/Three-Phase V-I Measurement  VoltageMeasurement=no  SetLabelV=on  LabelV=Vabc_NEM7  Vpu=on  VpuLL=off  CurrentMeasurement=no  SetLabelI=off  LabelI=A1  Ipu=off  Pbase=100e6  Vbase=735e3  OutputType=Magnitude  PhasorSimulation=off  PSBequivalent=0
  Regulators1 : Subsystem
  Regulators2 : Subsystem
  Regulators3 : Subsystem
  Regulators4 : Subsystem
  MTLa : PMIOPort  Port=1  Side=Right
  MTLb : PMIOPort  Port=2  Side=Right
  MTLc : PMIOPort  Port=3  Side=Right
  CHM7a : PMIOPort  Port=4  Side=Right
  CHM7b : PMIOPort  Port=5  Side=Right
  CHM7c : PMIOPort  Port=6  Side=Right
  wires:
  Regulators2/1(Pm) -> LG3_2200 MVA/1
  Regulators4/2(Vf) -> LG4-2700 MVA/2
  Regulators4/1(Pm) -> LG4-2700 MVA/1
  Regulators3/2(Vf) -> LG31-200 MVA/2
  Regulators3/1(Pm) -> LG31-200 MVA/1
  Regulators2/2(Vf) -> LG3_2200 MVA/2
  LG3_2200 MVA/1 -> Regulators2/1(m)
  Regulators1/1(Pm) -> LG2_5500 MVA/1
  Regulators1/2(Vf) -> LG2_5500 MVA/2
  LG2_5500 MVA/1 -> Regulators1/1(m)
  LG31-200 MVA/1 -> Regulators3/1(m)
  LG4-2700 MVA/1 -> Regulators4/1(m)
  connections:
  LG2-NENI 3*279km/RConn1 -- "Cs NEM "/LConn1
  LG2-NENI 3*279km/RConn2 -- "Cs NEM "/LConn2
  LG2-NENI 3*279km/RConn3 -- "Cs NEM "/LConn3
  CHB-CHM 3*195km/RConn1 -- "Cs  CHMN "/LConn1
  CHB-CHM 3*195km/RConn2 -- "Cs  CHMN "/LConn2
  CHB-CHM 3*195km/RConn3 -- "Cs  CHMN "/LConn3
  Load Flow Bus2/LConn1 -- 2200 MVA 13.8 kV/735 kV/LConn1 -- LG3_2200 MVA/RConn1 -- 110 MW/LConn1
  2200 MVA 13.8 kV/735 kV/LConn2 -- LG3_2200 MVA/RConn2 -- 110 MW/LConn2
  2200 MVA 13.8 kV/735 kV/LConn3 -- LG3_2200 MVA/RConn3 -- 110 MW/LConn3
  Load Flow Bus1/LConn1 -- 200 MVA 13.8 kV/735 kV/LConn1 -- LG31-200 MVA/RConn1 -- 10 MW/LConn1
  200 MVA 13.8 kV/735 kV/LConn2 -- LG31-200 MVA/RConn2 -- 10 MW/LConn2
  200 MVA 13.8 kV/735 kV/LConn3 -- LG31-200 MVA/RConn3 -- 10 MW/LConn3
  Load Flow Bus6/LConn1 -- 2200 MVA 13.8 kV/735 kV/RConn1 -- 200 MVA 13.8 kV/735 kV/RConn1 -- LG3-LMO 104km/LConn1 -- LG3 660 Mvar/LConn1 -- LG2-LG3 155km/RConn1
  2200 MVA 13.8 kV/735 kV/RConn2 -- LG3 660 Mvar/LConn2 -- LG2-LG3 155km/RConn2 -- 200 MVA 13.8 kV/735 kV/RConn2 -- LG3-LMO 104km/LConn2
  LG3-LMO 104km/RConn1 -- LMO7/RConn1 -- LG4-LMO 3*118km/RConn1 -- LMO 330 Mvar/LConn1
  LG3-LMO 104km/RConn2 -- LMO7/RConn2 -- LG4-LMO 3*118km/RConn2 -- LMO 330 Mvar/LConn2
  LG3-LMO 104km/RConn3 -- LMO7/RConn3 -- LG4-LMO 3*118km/RConn3 -- LMO 330 Mvar/LConn3
  LG4-LMO 3*118km/LConn1 -- LG4 660 Mvar/LConn1 -- 2700 MVA 13.8 kV/735 kV/RConn1 -- Load Flow Bus12/LConn1
  LG4-LMO 3*118km/LConn2 -- 2700 MVA 13.8 kV/735 kV/RConn2 -- LG4 660 Mvar/LConn2
  LG4 660 Mvar/LConn3 -- 2700 MVA 13.8 kV/735 kV/RConn3 -- LG4-LMO 3*118km/LConn3
  Load Flow Bus3/LConn1 -- LG4-2700 MVA/RConn1 -- 2700 MVA 13.8 kV/735 kV/LConn1 -- 135 MW/LConn1
  LG4-2700 MVA/RConn2 -- 2700 MVA 13.8 kV/735 kV/LConn2 -- 135 MW/LConn2
  LG4-2700 MVA/RConn3 -- 2700 MVA 13.8 kV/735 kV/LConn3 -- 135 MW/LConn3
  Load Flow Bus4/LConn1 -- 5500 MVA 13.8 kV/735 kV/LConn1 -- LG2_5500 MVA/RConn1 -- 275 MW/LConn1
  5500 MVA 13.8 kV/735 kV/LConn2 -- LG2_5500 MVA/RConn2 -- 275 MW/LConn2
  LG2_5500 MVA/RConn3 -- 5500 MVA 13.8 kV/735 kV/LConn3 -- 275 MW/LConn3
  5500 MVA 13.8 kV/735 kV/RConn1 -- LG2-NENI 3*279km/LConn1 -- LG2-LG3 155km/LConn1 -- LG2 660 Mvar/LConn1 -- Load Flow Bus5/LConn1
  LG2-LG3 155km/LConn2 -- 5500 MVA 13.8 kV/735 kV/RConn2 -- LG2-NENI 3*279km/LConn2 -- LG2 660 Mvar/LConn2
  LG2-LG3 155km/LConn3 -- 5500 MVA 13.8 kV/735 kV/RConn3 -- LG2-NENI 3*279km/LConn3 -- LG2 660 Mvar/LConn3
  "Cs NEM "/RConn1 -- NEM-ALB7/LConn1 -- Cs ALB/RConn1
  "Cs NEM "/RConn2 -- NEM-ALB7/LConn2 -- Cs ALB/RConn2
  "Cs NEM "/RConn3 -- NEM-ALB7/LConn3 -- Cs ALB/RConn3
  LMO7/LConn1 -- LMO-ALB 3*218km/LConn1
  LMO7/LConn2 -- LMO-ALB 3*218km/LConn2
  Load Flow Bus7/LConn1 -- LMO7/LConn3 -- LMO-ALB 3*218km/LConn3
  Cs ALB/LConn1 -- LMO-ALB 3*218km/RConn1
  Cs ALB/LConn2 -- LMO-ALB 3*218km/RConn2
  Cs ALB/LConn3 -- LMO-ALB 3*218km/RConn3
  200 MVA 13.8 kV/735 kV/RConn3 -- LG3-LMO 104km/LConn3 -- LG3 660 Mvar/LConn3 -- LG2-LG3 155km/RConn3 -- 2200 MVA 13.8 kV/735 kV/RConn3
  Load Flow Bus8/LConn1 -- NEM-ABI 6*236/LConn1 -- NEM-ALB7/RConn1 -- NEM-ALB 1980 Mvar/LConn1
  NEM-ALB 1980 Mvar/LConn2 -- NEM-ALB7/RConn2 -- NEM-ABI 6*236/LConn2
  NEM-ALB 1980 Mvar/LConn3 -- NEM-ALB7/RConn3 -- NEM-ABI 6*236/LConn3
  NEM-ABI 6*236/RConn1 -- "Cs ABI+CHB "/LConn1
  NEM-ABI 6*236/RConn2 -- "Cs ABI+CHB "/LConn2
  NEM-ABI 6*236/RConn3 -- "Cs ABI+CHB "/LConn3
  "Cs ABI+CHB "/RConn1 -- ABI-CHB7/LConn1
  "Cs ABI+CHB "/RConn2 -- ABI-CHB7/LConn2
  "Cs ABI+CHB "/RConn3 -- ABI-CHB7/LConn3
  Load Flow Bus9/LConn1 -- ABI+CHB 1320 Mvar/LConn1 -- CHB-CHM 3*195km/LConn1 -- ABI-CHB 3*271km/LConn1 -- ABI-CHB7/RConn1
  ABI-CHB 3*271km/LConn2 -- ABI-CHB7/RConn2 -- ABI+CHB 1320 Mvar/LConn2 -- CHB-CHM 3*195km/LConn2
  ABI-CHB 3*271km/LConn3 -- ABI-CHB7/RConn3 -- ABI+CHB 1320 Mvar/LConn3 -- CHB-CHM 3*195km/LConn3
  ABI-CHB 3*271km/RConn1 -- "Cs LVDN "/LConn1
  ABI-CHB 3*271km/RConn2 -- "Cs LVDN "/LConn2
  ABI-CHB 3*271km/RConn3 -- "Cs LVDN "/LConn3
  "Cs LVDN "/RConn1 -- LVD7/LConn1
  "Cs LVDN "/RConn2 -- LVD7/LConn2
  "Cs LVDN "/RConn3 -- LVD7/LConn3
  "Cs LVDS "/LConn1 -- LVD 990 Mvar/LConn1 -- Load Flow Bus10/LConn1 -- LVD7/RConn1
  "Cs LVDS "/LConn2 -- LVD7/RConn2 -- LVD 990 Mvar/LConn2
  "Cs LVDS "/LConn3 -- LVD7/RConn3 -- LVD 990 Mvar/LConn3
  "Cs LVDS "/RConn1 -- LVD-MTL 3*260km/LConn1
  "Cs LVDS "/RConn2 -- LVD-MTL 3*260km/LConn2
  "Cs LVDS "/RConn3 -- LVD-MTL 3*260km/LConn3
  MTLa/RConn1 -- LVD-MTL 3*260km/RConn1
  MTLb/RConn1 -- LVD-MTL 3*260km/RConn2
  MTLc/RConn1 -- LVD-MTL 3*260km/RConn3
  "Cs  CHMN "/RConn1 -- CHM7/LConn1
  "Cs  CHMN "/RConn2 -- CHM7/LConn2
  "Cs  CHMN "/RConn3 -- CHM7/LConn3
  CHM 1320Mvar/LConn2 -- CHM7/RConn2 -- CHM7b/RConn1
  Load Flow Bus11/LConn1 -- CHM 1320Mvar/LConn3 -- CHM7c/RConn1 -- CHM7/RConn3
  CHM7a/RConn1 -- CHM 1320Mvar/LConn1 -- CHM7/RConn1
